simulink model "ButtonLogic"  (R2023b)
settings: Solver=FixedStepDiscrete  StartTime=0.0  StopTime=inf  FixedStep=0.005  RelTol=1e-3  EnableMultiTasking=on
model workspace (MAT data in the model file):
  inSetButton = 0
undefined symbols (not defined in the file or in its folder): eStateName
libraries: simulink x5
(part 2 of 3)

== stateflow chart ButtonLogic/ButtonStates/buttonFlowChart ==
  state Flow [parallel]
    settings: executionOrder=3
    state ButtonTriggeredMenu
      state Menu
        state MainSubMenu
          (history)
          state LapTimer
            en:
            currentState = eStateName.LAP_TIMER;
            state LapTimerEntry
            state GreyedOut
            (default) -> (junction 222)
            LapTimerEntry -> 3149 : SET
            (junction 222) -> LapTimerEntry [order 1] : [rideMode == eRideMode.track]
            (junction 222) -> (junction 225) [order 2]
            (junction 225) -> GreyedOut
          state Motorcycle
            en:
            currentState = eStateName.MOTORCYCLE;
          state BikeInfo
            en:
            currentState = eStateName.BIKE_INFO;
          state TripInfo
            en:
            currentState = eStateName.TRIP_INFO;
          state CruiseControlMain
            en:
            currentState = eStateName.CRUISE_CONTROL;
          state NavigationMain
            en:
            currentState = eStateName.MAIN_NAVIGATION;
            state NavigationGreyedOut
            state NavigationVisible
            (default) -> (junction 1075)
            (junction 1075) -> NavigationGreyedOut [order 1] : [CCU_BT_Status == 0 || rideMode == eRideMode.track]
            (junction 1075) -> (junction 1080) [order 2]
            NavigationVisible -> 3067 : SET
            (junction 1080) -> NavigationVisible
          state HeatedGripsMain
            en:
            currentState = eStateName.HEATED_GRIPS;
          state AudioMain
            en:
            currentState = eStateName.AUDIO;
            state AudioVisible
            state AudioGreyedOut
            (default) -> (junction 1063)
            (junction 1063) -> AudioVisible [order 1] : [CCU_BT_Status == 1]
            AudioVisible -> 3021 : SET
            (junction 1063) -> (junction 1069) [order 2]
            (junction 1069) -> AudioGreyedOut
          state SettingsMain
            en:
            currentState = eStateName.SETTINGS;
            state SettingsGreyedOut
            state SettingsMenu
            (default) -> (junction 1245)
            (junction 1245) -> SettingsGreyedOut [order 1] : [vehSpeed>2.5]
            (junction 1245) -> (junction 1249) [order 2]
            (junction 1249) -> SettingsMenu
            SettingsMenu -> 3009 [order 2] : SET
            SettingsMenu -> 3011 [order 1] : [duration(up && down,msec)>=3000]
          (default) -> (junction 3141)
          (junction 3141) -> LapTimer [order 1] : [rideMode == eRideMode.track]
          (junction 3141) -> Motorcycle [order 2]
          (junction 3145) -> (junction 3141)
          LapTimer -> (junction 3151) [order 2] : UP
          (junction 4100) -> (junction 3151) [order 2]
          (junction 3151) -> (junction 3153)
          (junction 4100) -> LapTimer [order 1] : [rideMode == eRideMode.track]
          LapTimer -> Motorcycle [order 1] : DOWN
          Motorcycle -> (junction 4100) [order 1] : UP
          Motorcycle -> BikeInfo [order 2] : DOWN
          BikeInfo -> Motorcycle [order 1] : UP
          BikeInfo -> TripInfo [order 2] : DOWN
          TripInfo -> BikeInfo [order 1] : UP
          (junction 839) -> TripInfo
          CruiseControlMain -> (junction 839) [order 1] : UP
          (junction 194) -> (junction 839) [order 2]
          TripInfo -> (junction 154) [order 2] : DOWN
          (junction 154) -> CruiseControlMain [order 1] : [ECU_SL_Feature == 1 || ...
              | rideMode != eRideMode.track]
          (junction 194) -> CruiseControlMain [order 1] : [ECU_SL_Feature == 1]
          NavigationMain -> (junction 194) [order 2] : UP
          (junction 154) -> (junction 157) [order 2]
          (junction 189) -> (junction 194) [order 2]
          CruiseControlMain -> (junction 157) [order 2] : DOWN
          (junction 157) -> NavigationMain [order 1] : [CCU_Status == eCCUStatus.installed && CCU_TbT_Navigation_Feature == 1]
          (junction 189) -> NavigationMain [order 1] : [CCU_Status == eCCUStatus.installed && CCU_TbT_Navigation_Feature == 1]
          (junction 157) -> (junction 163) [order 2]
          HeatedGripsMain -> (junction 189) [order 2] : UP
          (junction 186) -> (junction 189) [order 2]
          NavigationMain -> (junction 163) [order 1] : DOWN
          (junction 163) -> HeatedGripsMain [order 1] : [Heated_Grips == 1 ]
              |  //Menu Settings/Heating/Heating Grip == Not available]
          (junction 163) -> (junction 171) [order 2]
          (junction 186) -> HeatedGripsMain [order 1] : [Heated_Grips == 1 ]
          Flow.ButtonTriggeredMenu.Menu.MainSubMenu.AudioMain -> (junction 186) [order 2] : UP
          (junction 183) -> (junction 186) [order 2] : [CCU_Status == eCCUStatus.notInstalled || CCU_Music_Feature == 0]
          HeatedGripsMain -> (junction 171) [order 1] : DOWN
          (junction 171) -> Flow.ButtonTriggeredMenu.Menu.MainSubMenu.AudioMain [order 1] : [CCU_Status == eCCUStatus.installed && CCU_Music_Feature == 1]
          (junction 171) -> (junction 177) [order 2]
          (junction 183) -> Flow.ButtonTriggeredMenu.Menu.MainSubMenu.AudioMain [order 1] : [CCU_Status == eCCUStatus.installed && CCU_Music_Feature == 1]
          (junction 4104) -> (junction 183) [order 2]
          (junction 181) -> (junction 183)
          Flow.ButtonTriggeredMenu.Menu.MainSubMenu.AudioMain -> (junction 177) [order 1] : DOWN
          (junction 3153) -> (junction 4104)
          (junction 4104) -> SettingsMain [order 1] : [vehSpeed<2.5]
          (junction 177) -> SettingsMain [order 1] : [vehSpeed<=2.5]
          SettingsMain -> (junction 181) [order 1] : UP
          (junction 177) -> (junction 3145) [order 2]
          SettingsMain -> (junction 3145) [order 2] : DOWN
        state Lap_TimerV1 [commented out]
          state LapTimerLoop [commented out]
            en:
            currentState = eStateName.RESET_LAPS;
            roundTimer = roundTimerData_arr[roundTimeCounter];
          state ResetLaps [commented out]
            state Keep [commented out]
              en:
              currentState = eStateName.KEEP;
            state Reset [commented out]
              en:
              currentState = eStateName.RESET;
              roundTimerData_arr[roundTimeCounter] =0;
              //updateRoundTimeData();
            (default) -> Flow.ButtonTriggeredMenu.Menu.Lap_TimerV1.ResetLaps.Keep [commented out]
            Flow.ButtonTriggeredMenu.Menu.Lap_TimerV1.ResetLaps.Keep -> Flow.ButtonTriggeredMenu.Menu.Lap_TimerV1.ResetLaps.Reset [commented out] : DOWN
            Flow.ButtonTriggeredMenu.Menu.Lap_TimerV1.ResetLaps.Reset -> Flow.ButtonTriggeredMenu.Menu.Lap_TimerV1.ResetLaps.Keep [commented out] : UP
          (default) -> Flow.ButtonTriggeredMenu.Menu.Lap_TimerV1.LapTimerLoop [commented out] : {roundTimeCounter = 0;
              | copyRoundTimeData();
              | updateRoundTimeData();}
          Flow.ButtonTriggeredMenu.Menu.Lap_TimerV1.LapTimerLoop -> (junction 237) [commented out] : DOWN
          (junction 237) -> (junction 240) [commented out] : [roundTimeCounter < BLU_MaxRndTimeLoopLim]
          (junction 240) -> (junction 239) [commented out] : {roundTimeCounter++;}
          (junction 237) -> (junction 239) [commented out]
          (junction 239) -> Flow.ButtonTriggeredMenu.Menu.Lap_TimerV1.LapTimerLoop [commented out]
          Flow.ButtonTriggeredMenu.Menu.Lap_TimerV1.LapTimerLoop -> (junction 245) [commented out] : UP
          (junction 245) -> (junction 247) [commented out] : [roundTimeCounter>0]
          (junction 247) -> (junction 249) [commented out] : {roundTimeCounter--;}
          (junction 245) -> (junction 249) [commented out]
          (junction 249) -> Flow.ButtonTriggeredMenu.Menu.Lap_TimerV1.LapTimerLoop [commented out]
          Flow.ButtonTriggeredMenu.Menu.Lap_TimerV1.LapTimerLoop -> Flow.ButtonTriggeredMenu.Menu.Lap_TimerV1.ResetLaps [commented out] : SET
          Flow.ButtonTriggeredMenu.Menu.Lap_TimerV1.ResetLaps -> Flow.ButtonTriggeredMenu.Menu.Lap_TimerV1.LapTimerLoop [commented out] : EXIT
        state NoQS
          en:
          QuickSelectorDbg = 1;
        state Lap_TimerV2
          state LapTimerLoop
            en:
            currentState = eStateName.RESET_LAPS;
          state RoundTimerMenu
            en:
            currentState = eStateName.RESET_LAPS_RND_TMR;
          state ResetLaps
            state ResetLapsMenu
              state Keep
                en:
                currentState = eStateName.RESETLAPS_KEEP;
              state Reset
                en:
                currentState = eStateName.RESETLAPS_RESET;
                //updateRoundTimeData();
              (default) -> Flow.ButtonTriggeredMenu.Menu.Lap_TimerV2.ResetLaps.ResetLapsMenu.Keep
              Flow.ButtonTriggeredMenu.Menu.Lap_TimerV2.ResetLaps.ResetLapsMenu.Keep -> Flow.ButtonTriggeredMenu.Menu.Lap_TimerV2.ResetLaps.ResetLapsMenu.Reset [order 1] : DOWN || UP
              Flow.ButtonTriggeredMenu.Menu.Lap_TimerV2.ResetLaps.ResetLapsMenu.Reset -> Flow.ButtonTriggeredMenu.Menu.Lap_TimerV2.ResetLaps.ResetLapsMenu.Keep [order 1] : DOWN || UP
            Flow.ButtonTriggeredMenu.Menu.Lap_TimerV2.ResetLaps.ResetLapsMenu.Keep -> (junction 3560) [order 2] : SET
            (junction 3560) -> 3554
            ResetLapsMenu -> 3554 : EXIT
            (junction 3565) -> 3554
            Flow.ButtonTriggeredMenu.Menu.Lap_TimerV2.ResetLaps.ResetLapsMenu.Reset -> (junction 3565) [order 2] : SET
                | {BLU_FnRLResetRndTmr();}
          (junction 4160) -> 3133
          RoundTimerMenu -> (junction 4160) [order 3] : EXIT
          Flow.ButtonTriggeredMenu.Menu.Lap_TimerV2.LapTimerLoop -> 3133 [order 2] : EXIT
          (default) -> (junction 3138)
          (junction 3138) -> Flow.ButtonTriggeredMenu.Menu.Lap_TimerV2.LapTimerLoop : {roundTimeCounter = 0;
              | copyRoundTimeData();
              | updateRoundTimeData();}
          3135 -> (junction 3138)
          (junction 4150) -> Flow.ButtonTriggeredMenu.Menu.Lap_TimerV2.LapTimerLoop
          (junction 4058) -> (junction 4150) [order 2]
          RoundTimerMenu -> (junction 4058) [order 1] : UP
          (junction 4058) -> (junction 4060) [order 1] : [BLU_RND_TMR_LOOP ==1]
          Flow.ButtonTriggeredMenu.Menu.Lap_TimerV2.LapTimerLoop -> (junction 4257) [order 4] : UP
          (junction 4257) -> RoundTimerMenu : [BLU_RND_TMR_LOOP ==1]
              | {BLU_FnLapTmrScrllUP();}
          (junction 4065) -> (junction 4058) [order 2]
          (junction 4060) -> (junction 4062) : {BLU_FnRLRndTmrUp();}
          (junction 4062) -> RoundTimerMenu
          Flow.ButtonTriggeredMenu.Menu.Lap_TimerV2.LapTimerLoop -> Flow.ButtonTriggeredMenu.Menu.Lap_TimerV2.ResetLaps [order 1] : SET
          3555 -> Flow.ButtonTriggeredMenu.Menu.Lap_TimerV2.LapTimerLoop
          Flow.ButtonTriggeredMenu.Menu.Lap_TimerV2.LapTimerLoop -> (junction 4052) [order 3] : DOWN
          (junction 4063) -> (junction 4062) : {BLU_FnRLRndTmrDwn();}
          (junction 4065) -> (junction 4063) [order 1] : [BLU_RND_TMR_LOOP ==1]
          RoundTimerMenu -> (junction 4065) [order 2] : DOWN
          (junction 4052) -> RoundTimerMenu : [BLU_RND_TMR_LOOP ==1]
              | {BLU_FnLapTmrScrllDOWN();}
        state MotorCycleSubMenu
          state MotorCycleSubMenu1
            (history)
            state RideMode
              en:
              currentState = eStateName.MOTORCYCLE_RIDEMODE;
            state ABS
              en:
              currentState = eStateName.MOTORCYCLE_ABS;
            state MTC
              en:
              currentState = eStateName.MOTORCYCLE_MTC;
            state LaunchControl
              en:
              currentState = eStateName.MOTORCYCLE_LAUNCHCONTROL;
            (junction 3116) -> RideMode
            (junction 3124) -> (junction 3116)
            RideMode -> (junction 3119) [order 3] : UP
            (junction 3119) -> (junction 3121)
            RideMode -> ABS [order 1] : DOWN
            ABS -> RideMode [order 1] : UP
            (junction 4113) -> ABS
            (junction 4111) -> (junction 4113) [order 2]
            MTC -> (junction 4113) [order 1] : UP
            ABS -> (junction 4107) [order 3] : DOWN
            (junction 4107) -> MTC [order 1] : [ABS_TC_MTC_Mode_Feature !=eTCMode.TCMode_OFF]
            (junction 3121) -> (junction 4246)
            (junction 4107) -> (junction 1612) [order 2]
            MTC -> (junction 1612) [order 2] : DOWN
            (junction 4111) -> MTC [order 1] : [ABS_TC_MTC_Mode_Feature !=eTCMode.TCMode_OFF]
            (junction 4246) -> (junction 4111) [order 2]
            (junction 4246) -> (junction 4248) [order 1] : [rideMode == eRideMode.rain && ...
                | ABS_Launch_Control_Feature == 1]
            LaunchControl -> (junction 4111) [order 1] : UP
            (junction 1612) -> LaunchControl [order 1] : [rideMode == eRideMode.rain && ...
                | ABS_Launch_Control_Feature == 1]
            (junction 1612) -> (junction 3551) [order 2]
            (junction 4248) -> LaunchControl
            (junction 3551) -> (junction 3124)
            LaunchControl -> (junction 3551) [order 3] : DOWN
          state RideModeSubMenu
            state RideModeSubMenu1
              (history)
              state Track
                en:
                currentState = eStateName.MC_RIDEMODE_TRACK;
              state Street
                en:
                currentState = eStateName.MC_RIDEMODE_STREET;
              state Rain
                en:
                currentState = eStateName.MC_RIDEMODE_RAIN;
              Track -> (junction 3105) [order 1]
              (junction 3112) -> Track
              (junction 3105) -> (junction 3107) [order 2] : DOWN
              (junction 3110) -> (junction 3112)
              Track -> Street [order 2] : UP
              Street -> Track [order 3] : DOWN
              Rain -> Street [order 1] : DOWN
              Street -> Rain [order 2] : UP
              (junction 3107) -> Rain
              Rain -> (junction 3110) [order 3] : UP
            state TrackCloseThrottle
              en:
              currentState = eStateName.MC_CLOSETHROTTLE;
            state KillSwitch
              en:
              currentState = eStateName.MC_DEACTIVATE_KILLSWITCH;
            state StreetCloseThrottle
              en:
              currentState = eStateName.MC_CLOSETHROTTLE;
            state RainCloseThrottle
              en:
              currentState = eStateName.MC_CLOSETHROTTLE;
            (junction 3105) -> (junction 1639) [order 1] : SET
            (junction 1639) -> (junction 2456) [order 1] : [killSwitch == eSwitch.closed]
            (junction 2456) -> TrackCloseThrottle : {DASH_TC_Mode_Request = 0;
                | DASH_Drive_Mode_Request = 0;}
            (junction 1639) -> KillSwitch [order 2]
            TrackCloseThrottle -> (junction 1665) [order 2] : after(5,sec)
            TrackCloseThrottle -> (junction 1664) [order 1] : after(500,msec)
            KillSwitch -> (junction 1659) : [after(1,sec)]
            (junction 1665) -> (junction 1659)
            (junction 1664) -> (junction 1665) : [ABS_TC_Mode_Response == 0 && ...
                | ECU_Drive_Mode_Response == 0]
                | {rideMode = eRideMode.track;}
            (junction 1659) -> (junction 1680)
            (junction 1651) -> KillSwitch [order 2]
            2646 -> (junction 2143)
            (junction 2143) -> Street
            2655 -> (junction 2143)
            Street -> (junction 1651) [order 1] : SET
            (junction 1651) -> (junction 2458) [order 1] : [killSwitch == eSwitch.closed]
            (junction 2458) -> StreetCloseThrottle : {DASH_TC_Mode_Request = 0;
                | DASH_Drive_Mode_Request = 0;}
            StreetCloseThrottle -> (junction 2611) [order 1] : after(500,msec)
            (junction 1654) -> (junction 1651) [order 2]
            (junction 2611) -> (junction 2615) : [ABS_TC_Mode_Response == 0 && ...
                | ECU_Drive_Mode_Response == 0]
                | {rideMode = eRideMode.street;}
            StreetCloseThrottle -> (junction 1677) [order 2] : after(5,sec)
            (junction 1677) -> (junction 1680)
            (junction 2615) -> (junction 1677)
            (junction 1680) -> 2653
            RainCloseThrottle -> (junction 1677) [order 2] : after(5,sec)
            (junction 2613) -> (junction 2615) : [ABS_TC_Mode_Response == 2 && ...
                | ECU_Drive_Mode_Response == 2]
                | {rideMode = eRideMode.rain;}
            RainCloseThrottle -> (junction 2613) [order 1] : after(500,msec)
            Rain -> (junction 1654) [order 2] : SET
            (junction 1654) -> (junction 2459) [order 1] : [killSwitch == eSwitch.closed]
            (junction 2459) -> RainCloseThrottle : {DASH_TC_Mode_Request = 2;
                | DASH_Drive_Mode_Request = 2;}
            RideModeSubMenu1 -> 2653 : EXIT
          state ABSSubMenu
            state ABSMenu1
              (history)
              state ABSRoad
                en:
                currentState = eStateName.ABS_ROAD;
              state ABSSuperMoto
                en:
                currentState = eStateName.ABS_SUPERMOTO;
              ABSRoad -> (junction 1706) [order 1] : DOWN || UP
              ABSSuperMoto -> ABSRoad [order 1] : DOWN || UP
              (junction 1706) -> ABSSuperMoto : [ABS_Mode_Feature == 1]
            state SetABStoRoad
              en:
              DASH_ABS_Mode_Request = eABSMode.road;
            state SetABStoSupermoto
              en:
              DASH_ABS_Mode_Request = eABSMode.supermoto;
            2154 -> (junction 2156)
            SetABStoRoad -> (junction 2669) [order 1] : after(500,msec)
            ABSRoad -> SetABStoRoad [order 2] : SET
            (junction 2156) -> ABSRoad
            (junction 2669) -> (junction 2550) : [ABS_ABS_Mode_Response == eABSMode.road]
            2642 -> (junction 2156)
            SetABStoRoad -> (junction 2553) [order 2] : after(5,sec)
            (junction 2550) -> (junction 2553)
            ABSMenu1 -> 2636 : EXIT
            (junction 2553) -> 2636
            SetABStoSupermoto -> (junction 2553) [order 2] : after(5,sec)
            (junction 2671) -> (junction 2550) : [ABS_ABS_Mode_Response == eABSMode.supermoto]
            SetABStoSupermoto -> (junction 2671) [order 1] : after(500,msec)
            ABSSuperMoto -> SetABStoSupermoto [order 2] : SET
          state MTCSubMenu
            state MTCMenuOptions
              (history)
              state MTC_Off
                en:
                currentState = eStateName.MTCMODE_OFF;
              state MTC_On
                en:
                currentState = eStateName.MTCMODE_ON;
              (default) -> MTC_Off
              MTC_Off -> MTC_On [order 1] : DOWN || UP
              MTC_On -> MTC_Off [order 1] : DOWN || UP
            state MTC_Message
              en:
              currentState = eStateName.MTC_KEEP_OFF_PRESS;
            state MTC_Release
              en:
              currentState = eStateName.MTC_OFF_RELEASE;
            state MTC_Message1
              en:
              currentState = eStateName.MTC_KEEP_ON_PRESS;
            state MTC_Release1
              en:
              currentState = eStateName.MTC_ON_RELEASE;
            2163 -> (junction 2165)
            (junction 2165) -> (junction 1732)
            (junction 1732) -> (junction 1734) [order 1] : [ABS_TC_MTC_Mode_Feature == eTCMode.TCMode_TC || ...
                | ABS_TC_MTC_Mode_Feature == eTCMode.TCMode_TC_Demo ]
            (junction 1732) -> (junction 1739) [order 2]
            2630 -> (junction 2165)
            (junction 1734) -> (junction 1741) : {currentState = eStateName.MTCMODE_TC;}
            (junction 1739) -> (junction 1741) : {currentState = eStateName.MTCMODE_MTC;}
            (junction 1741) -> MTCMenuOptions
            MTC_Off -> MTC_Message [order 2] : [set]
            MTC_Message -> MTC_Release [order 2] : after(3,sec)
            MTC_Message -> (junction 2545) [order 1] : [!set]
            MTC_Release -> (junction 1761) : [!set]
                | {DASH_MTC_Off_Switch = eButton.pressed;}
            MTCMenuOptions -> 2623 : EXIT
            (junction 2545) -> 2623
            (junction 1761) -> (junction 2545)
            MTC_Message1 -> (junction 2545) [order 1] : [!set]
            MTC_Release1 -> (junction 1761) : [!set]
                | {DASH_MTC_Off_Switch = eButton.released;}
            MTC_On -> MTC_Message1 [order 2] : [set]
            MTC_Message1 -> MTC_Release1 [order 2] : after(3,sec)
          state LaunchControlSubMenu
            state LaunchControlSubMenu1
              (history)
              state LaunchControlON
                en:
                currentState = eStateName.MC_LAUNCHCONTROL_ON;
              state LaunchControlOFF
                en:
                currentState = eStateName.MC_LAUNCHCONTROL_OFF;
              LaunchControlON -> LaunchControlOFF [order 2] : DOWN || UP
              LaunchControlOFF -> LaunchControlON [order 1] : DOWN || UP
            2616 -> LaunchControlON
            LaunchControlON -> (junction 1785) [order 1] : SET
            (junction 1785) -> (junction 1789) : {BLU_FnLaunchControlON();}
            (junction 1787) -> (junction 1789) : {BLU_FnLaunchControlOFF();}
            (junction 1789) -> 2618
            LaunchControlOFF -> (junction 1787) [order 2] : SET
            LaunchControlSubMenu1 -> 2618 : EXIT
          3127 -> (junction 3116)
          RideMode -> 2656 [order 2] : SET
          2649 -> 2647
          2654 -> (junction 2659)
          (junction 2659) -> (junction 2639)
          ABS -> 2643 [order 2] : SET
          2287 -> 2155
          2637 -> (junction 2639)
          (junction 2639) -> (junction 2633)
          MotorCycleSubMenu1 -> 3130 : EXIT
          (junction 1728) -> 2631 : [ABS_TC_MTC_Mode_Feature == eTCMode.TCMode_TC || ...
              | ABS_TC_MTC_Mode_Feature == eTCMode.TCMode_MTC || ...
              | ABS_TC_MTC_Mode_Feature == eTCMode.TCMode_TC_Demo || ...
              | ABS_TC_MTC_Mode_Feature == eTCMode.TCMode_MTC_Demo ]
          MTC -> (junction 1728) [order 3] : SET
          2290 -> 2164
          2624 -> (junction 2633)
          (junction 2633) -> (junction 2662)
          (junction 2662) -> MotorCycleSubMenu1
          2619 -> (junction 2662)
          LaunchControl -> 2617 [order 2] : SET
        state BikeInfoSubMenu
          state BikeInfoSubMenuMain
            state WaterTemp
              en:
              currentState = eStateName.WATER_TEMPERATURE;
            state FuelRange
              en:
              currentState = eStateName.FUEL_RANGE;
            state Battery
              en:
              currentState = eStateName.BATTERY;
            state Odometer
              en:
              currentState = eStateName.ODOMETER;
            state Service
              en:
              currentState = eStateName.SERVICE;
            state Warnings
              en:
              currentState = eStateName.WARNINGS;
            (default) -> (junction 3096)
            WaterTemp -> (junction 3088) [order 2] : UP
            (junction 3096) -> WaterTemp
            (junction 3094) -> (junction 3096)
            (junction 3088) -> (junction 3090)
            WaterTemp -> FuelRange [order 1] : DOWN
            FuelRange -> WaterTemp [order 2] : UP
            FuelRange -> Battery [order 1] : DOWN
            Battery -> FuelRange [order 2] : UP
            Battery -> Odometer [order 1] : DOWN
            Odometer -> Battery [order 2] : UP
            Odometer -> Service [order 1] : DOWN
            Service -> Odometer [order 2] : UP
            Service -> Warnings [order 1] : DOWN
            Warnings -> Service [order 1] : UP
            (junction 3090) -> Warnings
            Warnings -> (junction 3094) [order 3] : DOWN
          state WarningsSubMenu
            en:
            currentState = eStateName.WARNINGS_MENU;
          3099 -> BikeInfoSubMenuMain
          4047 -> BikeInfoSubMenuMain
          BikeInfoSubMenuMain -> 3102 : EXIT
          WarningsSubMenu -> (junction 454) [order 2] : UP
          (junction 454) -> (junction 456) : {BLU_FnBIWarningsUp();}
          WarningsSubMenu -> (junction 3090) [order 1] : EXIT
          (junction 456) -> WarningsSubMenu
          (junction 460) -> (junction 456) : {BLU_FnBIWarningsDwn();}
          Warnings -> WarningsSubMenu [order 2] : SET
          WarningsSubMenu -> (junction 460) [order 3] : DOWN
        state TripInfoSubMenu
          state TripInfoSubMenuMain
            (history)
            state TRIP1
              en:
              currentState = eStateName.TRIP_INFO_TRIP_1;
            state TRIP2
              en:
              currentState = eStateName.TRIP_INFO_TRIP_2;
            TRIP1 -> TRIP2 [order 1] : DOWN || UP
            TRIP2 -> TRIP1 [order 1] : DOWN || UP
          state Trip1
            state Trip1SubMenu
              state SetAsOverview
                en:
                currentState = eStateName.TRIP_1_SET_AS_OVERVIEW;
              state ResetTrip
                en:
                currentState = eStateName.TRIP_1_RESET_TRIP;
              Flow.ButtonTriggeredMenu.Menu.TripInfoSubMenu.Trip1.Trip1SubMenu.SetAsOverview -> (junction 2202) [order 2] : SET
                  | {BLU_FnTISetAsOvwTrip1();}
              (junction 2202) -> (junction 398)
              Flow.ButtonTriggeredMenu.Menu.TripInfoSubMenu.Trip1.Trip1SubMenu.SetAsOverview -> Flow.ButtonTriggeredMenu.Menu.TripInfoSubMenu.Trip1.Trip1SubMenu.ResetTrip [order 1] : DOWN || UP
              Flow.ButtonTriggeredMenu.Menu.TripInfoSubMenu.Trip1.Trip1SubMenu.ResetTrip -> Flow.ButtonTriggeredMenu.Menu.TripInfoSubMenu.Trip1.Trip1SubMenu.SetAsOverview [order 1] : DOWN || UP
              Flow.ButtonTriggeredMenu.Menu.TripInfoSubMenu.Trip1.Trip1SubMenu.ResetTrip -> (junction 398) [order 2] : SET
                  | {BLU_FnTIResetTrip1();}
            2176 -> (junction 2175)
            (junction 2175) -> Flow.ButtonTriggeredMenu.Menu.TripInfoSubMenu.Trip1.Trip1SubMenu.SetAsOverview
            (default) -> (junction 2175)
            (junction 398) -> 3935
            Trip1SubMenu -> 3935 : EXIT
          state Trip2
            state Trip2SubMenu
              state SetAsOverview
                en:
                currentState = eStateName.TRIP_2_SET_AS_OVERVIEW;
              state ResetTrip
                en:
                currentState = eStateName.TRIP_2_RESET_TRIP;
              Flow.ButtonTriggeredMenu.Menu.TripInfoSubMenu.Trip2.Trip2SubMenu.SetAsOverview -> (junction 410) [order 2] : SET
                  | {BLU_FnTISetAsOvwTrip2();}
              (junction 2205) -> (junction 410)
              Flow.ButtonTriggeredMenu.Menu.TripInfoSubMenu.Trip2.Trip2SubMenu.SetAsOverview -> Flow.ButtonTriggeredMenu.Menu.TripInfoSubMenu.Trip2.Trip2SubMenu.ResetTrip [order 1] : DOWN || UP
              Flow.ButtonTriggeredMenu.Menu.TripInfoSubMenu.Trip2.Trip2SubMenu.ResetTrip -> Flow.ButtonTriggeredMenu.Menu.TripInfoSubMenu.Trip2.Trip2SubMenu.SetAsOverview [order 1] : DOWN || UP
              Flow.ButtonTriggeredMenu.Menu.TripInfoSubMenu.Trip2.Trip2SubMenu.ResetTrip -> (junction 2205) [order 2] : SET
                  | {BLU_FnTIResetTrip2();}
            (junction 3943) -> 3940
            Trip2SubMenu -> 3940 : EXIT
            (junction 410) -> (junction 3943)
            2209 -> (junction 2212)
            (default) -> (junction 2212)
            (junction 2212) -> Flow.ButtonTriggeredMenu.Menu.TripInfoSubMenu.Trip2.Trip2SubMenu.SetAsOverview
          TRIP1 -> Trip1 [order 2] : SET
          2269 -> 2177
          3082 -> TRIP1
          3936 -> (junction 3946)
          (junction 3946) -> TripInfoSubMenuMain
          3941 -> (junction 3946)
          TripInfoSubMenuMain -> 3080 : EXIT
          TRIP2 -> Trip2 [order 2] : SET
          2273 -> 2210
        state CruiseCtrlSubMenu
          note: Invisible when ECU_CC_Feature == 0
          note: Invisible when ECU_CC_Feature == 1
          state Mode
            en:
            currentState = eStateName.MODE_CC;
          state SpeedLimiter
            en:
            currentState = eStateName.SPEED_LIMITER;
          state SpeedLimiterSubMenu
            (history)
            state SL_ON
              en:
              currentState = eStateName.SPEED_LIMITER_ON;
            state SL_OFF
              en:
              currentState = eStateName.SPEED_LIMITER_OFF;
            (default) -> SL_ON
            SL_ON -> SL_OFF [order 1] : DOWN || UP
            SL_OFF -> SL_ON [order 1] : DOWN || UP
          state ECU_SL_StatusCheck1
            state DashSLONCheck
              en:
              currentState = eStateName.SPEED_LIMITER_ONCHECK;
            state DashSLOFFCheck
              en:
              currentState = eStateName.SPEED_LIMITER_OFFCHECK;
          state ModeSubMenu
            (history)
            state CruiseControlMode1
              en:
              currentState = eStateName.CRUISE_CONTROL_MODE;
            state SpeedLimiterMode
              en:
              currentState = eStateName.SPEED_LIMITER_MODE;
            (default) -> CruiseControlMode1
            CruiseControlMode1 -> SpeedLimiterMode [order 1] : DOWN || UP
            SpeedLimiterMode -> CruiseControlMode1 [order 1] : DOWN || UP
          state ECU_SL_StatusCheck2
            state DashCruiseCtrlChck
              en:
              currentState = eStateName.CRUISE_CONTROL_CHECK;
            state DashSpeedLmtrChck
              en:
              currentState = eStateName.SPEED_LIMITER_MODE_CHECK;
          3072 -> (junction 481)
          (default) -> (junction 481)
          (junction 481) -> SpeedLimiter [order 2]
          (junction 481) -> Mode [order 1] : [ECU_CC_Feature == 1]
          2266 -> (junction 481)
          SpeedLimiter -> SpeedLimiterSubMenu [order 1] : SET
          (junction 4251) -> SpeedLimiter
          SpeedLimiter -> 3070 [order 2] : EXIT
          Mode -> (junction 490) [order 1] : EXIT
          (junction 4253) -> Mode
          Mode -> ModeSubMenu [order 2] : SET
          (junction 4189) -> (junction 4185)
          (junction 4185) -> (junction 4169)
          (junction 4169) -> (junction 4253)
          (junction 490) -> 3070
          ECU_SL_StatusCheck2 -> (junction 4185) [order 2] : [after(5,sec)]
          ECU_SL_StatusCheck2 -> (junction 4189) [order 1] : EXIT
          ModeSubMenu -> (junction 4253) : EXIT
          (junction 550) -> (junction 4169)
          SpeedLimiterSubMenu -> (junction 4251) : EXIT
          (junction 4192) -> (junction 4251)
          (junction 4194) -> (junction 4192)
          (junction 512) -> (junction 4251)
          ECU_SL_StatusCheck1 -> (junction 4192) [order 2] : [after(5,sec)]
          ECU_SL_StatusCheck1 -> (junction 4194) [order 1] : EXIT
          CruiseControlMode1 -> DashCruiseCtrlChck [order 2] : SET
              | {DASH_SL_Switch =1;}
          SL_ON -> DashSLONCheck [order 2] : SET
              | {DASH_SL_Switch =1;}
          DashCruiseCtrlChck -> (junction 550) : [ ECU_SL_Status == 0]
              | {BLU_FnCCSwtONCrsCtrl();}
          DashSLONCheck -> (junction 512) : [ ECU_SL_Status == 1]
              | {BLU_FnCCSwtONSpdLmtr();}
          (junction 540) -> (junction 550)
          (junction 523) -> (junction 512)
          SL_OFF -> DashSLOFFCheck [order 2] : SET
              | {DASH_SL_Switch =1;}
          SpeedLimiterMode -> DashSpeedLmtrChck [order 2] : SET
              | {DASH_SL_Switch =1;}
          DashSLOFFCheck -> (junction 523) : [ ECU_SL_Status == 0]
              | {BLU_FnCCSwtOFFSpdLmtr();}
          DashSpeedLmtrChck -> (junction 540) : [ ECU_SL_Status == 1]
              | {BLU_FnCCSwtONSpdLmtr();}
        state NavigationVolSubMenu
          state NavGroup
            (history)
            state Volume
              en:
              currentState = eStateName.NAVIGATION_VOLUME;
            state Navigation
              en:
              currentState = eStateName.NAVIGATION;
            (default) -> Volume
            Volume -> Navigation [order 1] : DOWN || UP
            Navigation -> Volume [order 1] : DOWN || UP
          state VolumeSubMenu
            en:
            currentState = eStateName.NAVIGATION_VOL_SUB_MN;
          state NavigationSubMenu
            (history)
            state Nav_ON
              en:
              currentState = eStateName.NAVIGATION_ON;
            state Nav_OFF
              en:
              currentState = eStateName.NAVIGATION_OFF;
            (default) -> Nav_ON
            Nav_ON -> Nav_OFF [order 1] : DOWN || UP
            Nav_OFF -> Nav_ON [order 1] : DOWN || UP
          2665 -> (junction 2301)
          VolumeSubMenu -> (junction 566) [order 2] : UP
          (junction 566) -> (junction 568) : {BLU_FnNavVolUp();}
          (junction 568) -> VolumeSubMenu
          (junction 2301) -> NavGroup
          (junction 569) -> (junction 568) : {BLU_FnNavVolDwn();}
          Volume -> VolumeSubMenu [order 2] : SET
          3064 -> (junction 2301)
          VolumeSubMenu -> (junction 569) [order 3] : DOWN
          VolumeSubMenu -> (junction 3057) [order 1] : EXIT
          (junction 3950) -> (junction 3057)
          (junction 3057) -> NavGroup
          (junction 2393) -> (junction 3950)
          NavigationSubMenu -> (junction 3057) : EXIT
          NavGroup -> 3062 : EXIT
          Navigation -> NavigationSubMenu [order 2] : SET
          Nav_ON -> (junction 2389) [order 2] : SET
          (junction 2389) -> (junction 2393) : {navigationStatus = eFeatureStatus.enabled;
              | BLU_FnNavigationStatus(navigationStatus);}
          (junction 2391) -> (junction 2393) : {navigationStatus = eFeatureStatus.disabled;
              | BLU_FnNavigationStatus(navigationStatus);}
          Nav_OFF -> (junction 2391) [order 2] : SET
        state HeatedGripsSubMenu
          state HeatedGripsMenuGrp
            (history)
            state HeatedGripsOFF
              en:
              currentState = eStateName.HEATED_GRIPS_OFF;
              HeatedGripsMode = eHeatedGripsMode.OFF;
            state HeatedGripsMAXIMUM
              en:
              currentState = eStateName.HEATED_GRIPS_MAXIMUM;
              HeatedGripsMode = eHeatedGripsMode.MAXIMUM;
            state HeatedGripsMEDIUM
              en:
              currentState = eStateName.HEATED_GRIPS_MEDIUM;
              HeatedGripsMode = eHeatedGripsMode.MEDIUM;
            state HeatedGripsMINIMUM
              en:
              currentState = eStateName.HEATED_GRIPS_MINIMUM;
              HeatedGripsMode = eHeatedGripsMode.MINIMUM;
            HeatedGripsOFF -> (junction 3042) [order 2] : UP
            (junction 3042) -> (junction 3044)
            (junction 3049) -> HeatedGripsOFF
            (junction 3047) -> (junction 3049)
            HeatedGripsOFF -> HeatedGripsMAXIMUM [order 1] : DOWN
            HeatedGripsMAXIMUM -> HeatedGripsOFF [order 1] : UP
            HeatedGripsMAXIMUM -> HeatedGripsMEDIUM [order 2] : DOWN
            HeatedGripsMEDIUM -> HeatedGripsMAXIMUM [order 1] : UP
            HeatedGripsMEDIUM -> HeatedGripsMINIMUM [order 2] : DOWN
            HeatedGripsMINIMUM -> HeatedGripsMEDIUM [order 1] : UP
            (junction 3044) -> HeatedGripsMINIMUM
            HeatedGripsMINIMUM -> (junction 3047) [order 2] : DOWN
          2319 -> (junction 3049)
          3052 -> (junction 3049)
          HeatedGripsMenuGrp -> 3055 [order 1] : EXIT
          (junction 3813) -> 3055 : {BLU_FnSetHeatedGripsMode(HeatedGripsMode);}
          HeatedGripsMenuGrp -> (junction 3813) [order 2] : SET
        state AudioSubMenu
          state AudioMain
            en:
            currentState = eStateName.AUDIO_SUB_MENU;
          Flow.ButtonTriggeredMenu.Menu.AudioSubMenu.AudioMain -> (junction 622) [order 1] : SET
          (junction 622) -> (junction 624) : {BLU_FnAudioTglPlayPause();}
          (junction 624) -> (junction 634)
          2221 -> (junction 2223)
          Flow.ButtonTriggeredMenu.Menu.AudioSubMenu.AudioMain -> (junction 626) [order 2] : longUP
          (junction 626) -> (junction 634) : {BLU_FnAudioVolUp();}
          (junction 634) -> (junction 636)
          Flow.ButtonTriggeredMenu.Menu.AudioSubMenu.AudioMain -> (junction 628) [order 3] : longDOWN
          (junction 628) -> (junction 636) : {BLU_FnAudioVolDwn();}
          (junction 2223) -> Flow.ButtonTriggeredMenu.Menu.AudioSubMenu.AudioMain
          3017 -> (junction 2223)
          (junction 636) -> (junction 640)
          Flow.ButtonTriggeredMenu.Menu.AudioSubMenu.AudioMain -> (junction 630) [order 4] : UP
          (junction 630) -> (junction 640) : {BLU_FnAudioNextTrack();}
          (junction 640) -> (junction 643)
          Flow.ButtonTriggeredMenu.Menu.AudioSubMenu.AudioMain -> 3014 [order 6] : EXIT
          Flow.ButtonTriggeredMenu.Menu.AudioSubMenu.AudioMain -> (junction 632) [order 5] : DOWN
          (junction 632) -> (junction 643) : {BLU_FnAudioPrevTrack();}
          (junction 643) -> (junction 646)
          (junction 646) -> Flow.ButtonTriggeredMenu.Menu.AudioSubMenu.AudioMain
        state SettingsSubMenu
          state SettingsMenuScreens
            (history)
            state Favourites
              en:
              currentState = eStateName.FAVOURITES;
            state QuickSelector
              en:
              currentState = eStateName.QUICK_SELECTOR;
            state Connectivity
              en:
              currentState = eStateName.CONNECTIVITY;
            state QuickShifter
              en:
              currentState = eStateName.QUICK_SHIFTER;
            state ShiftLight
              en:
              currentState = eStateName.SHIFT_LIGHT;
            state ClockDate
              en:
              currentState = eStateName.CLOCK_DATE_MN;
            state Units
              en:
              currentState = eStateName.UNITS;
            state Language
              en:
              currentState = eStateName.LANGUAGE;
            state HeatedGripsSettingsMenu
              en:
              currentState = eStateName.HEATED_GRIPS_SETTINGS_MN;
            state ExtraFunctions
              en:
              currentState = eStateName.EXTRA_FUNCTIONS;
            (default) -> (junction 2702)
            (junction 2702) -> Favourites
            (junction 2710) -> (junction 2702)
            Favourites -> (junction 2705) [order 3] : UP
            (junction 2705) -> (junction 2707)
            Favourites -> QuickSelector [order 2] : DOWN
            QuickSelector -> Favourites [order 2] : UP
            (junction 722) -> QuickSelector
            (junction 1102) -> (junction 722) [order 2] : UP
            (junction 719) -> (junction 722) [order 2]
            QuickSelector -> (junction 668) [order 3] : DOWN
            Connectivity -> (junction 1102) [order 1]
            (junction 668) -> Connectivity [order 1] : [CCU_Status == eCCUStatus.installed]
            (junction 668) -> (junction 671) [order 2]
            Connectivity -> (junction 671) [order 2] : DOWN
            (junction 719) -> Connectivity [order 1] : [CCU_Status == eCCUStatus.installed]
            (junction 1134) -> (junction 719) [order 1] : UP
            (junction 711) -> (junction 719) [order 2]
            QuickShifter -> (junction 1134) [order 1]
            (junction 711) -> QuickShifter [order 1] : [ECU_Quickshifter_Feature != 0]
            (junction 671) -> QuickShifter [order 1] : [ECU_Quickshifter_Feature != 0]
            (junction 709) -> (junction 711)
            (junction 671) -> (junction 676) [order 2]
            QuickShifter -> (junction 676) [order 2] : DOWN
            Flow.ButtonTriggeredMenu.Menu.SettingsSubMenu.SettingsMenuScreens.ShiftLight -> (junction 709) [order 2] : UP
            (junction 676) -> Flow.ButtonTriggeredMenu.Menu.SettingsSubMenu.SettingsMenuScreens.ShiftLight
            Flow.ButtonTriggeredMenu.Menu.SettingsSubMenu.SettingsMenuScreens.ShiftLight -> (junction 713) [order 1] : DOWN
            (junction 713) -> ClockDate
            (junction 715) -> Flow.ButtonTriggeredMenu.Menu.SettingsSubMenu.SettingsMenuScreens.ShiftLight [order 1] : UP
            ClockDate -> (junction 715) [order 1]
            ClockDate -> Units [order 2] : DOWN
            Units -> ClockDate [order 1] : UP
            Units -> Language [order 2] : DOWN
            Language -> Units [order 1] : UP
            (junction 706) -> Language
            HeatedGripsSettingsMenu -> (junction 706) [order 1] : UP
            (junction 703) -> (junction 706) [order 2]
            Language -> (junction 699) [order 2] : DOWN
            (junction 699) -> HeatedGripsSettingsMenu [order 1] : [Heated_Grips]
            (junction 699) -> ExtraFunctions [order 2]
            (junction 703) -> HeatedGripsSettingsMenu [order 1] : [Heated_Grips]
            (junction 702) -> (junction 703)
            HeatedGripsSettingsMenu -> ExtraFunctions [order 2] : DOWN
            (junction 2707) -> ExtraFunctions
            ExtraFunctions -> (junction 2710) [order 3] : DOWN
            ExtraFunctions -> (junction 702) [order 1] : UP
          state FavoritesSubMenu
            state FavoritesSlotsMenu
              state FavoritesSlot1
                en:
                currentState = eStateName.FAVORITES_SLOT_1;
              state FavoritesSlot2
                en:
                currentState = eStateName.FAVORITES_SLOT_2;
              state FavoritesSlot3
                en:
                currentState = eStateName.FAVORITES_SLOT_3;
              state FavoritesSlot4
                en:
                currentState = eStateName.FAVORITES_SLOT_4;
              (default) -> (junction 2990)
              (junction 2990) -> FavoritesSlot1
              (junction 2988) -> (junction 2990)
              FavoritesSlot1 -> (junction 2995) [order 3] : UP
              (junction 2995) -> (junction 2997)
              FavoritesSlot1 -> FavoritesSlot2 [order 1] : DOWN
              FavoritesSlot2 -> FavoritesSlot1 [order 2] : UP
              FavoritesSlot2 -> FavoritesSlot3 [order 3] : DOWN
              FavoritesSlot3 -> FavoritesSlot2 [order 1] : UP
              FavoritesSlot3 -> FavoritesSlot4 [order 2] : DOWN
              FavoritesSlot4 -> FavoritesSlot3 [order 1] : UP
              (junction 2997) -> FavoritesSlot4
              FavoritesSlot4 -> (junction 2988) [order 3] : DOWN
            state Slot1Menu
              state Slot1FavoritesMenu
                (history)
                state Slot1TripDistance1
                  en:
                  currentState = eStateName.FAVORITES_TRIP_DISTANCE_1;
                state Slot1AverageSpeed1
                  en:
                  currentState = eStateName.FAVORITES_AVERAGE_SPEED_1;
                state Slot1AverageFuelCons1
                  en:
                  currentState = eStateName.FAVORITES_AVERAGE_FUEL_CONS_1;
                state Slot1TripTime1
                  en:
                  currentState = eStateName.FAVORITES_TRIP_TIME_1;
                state Slot1AverageTripDistance2
                  en:
                  currentState = eStateName.FAVORITES_TRIP_DISTANCE_2;
                state Slot1AverageSpeed2
                  en:
                  currentState = eStateName.FAVORITES_AVERAGE_SPEED_2;
                state Slot1AverageFuelCons2
                  en:
                  currentState = eStateName.FAVORITES_AVERAGE_FUEL_CONS_2;
                state Slot1TripTime2
                  en:
                  currentState = eStateName.FAVORITES_TRIP_TIME_2;
                state Slot1FuelRange
                  en:
                  currentState = eStateName.FAVORITES_FUEL_RANGE;
                state Slot1Date
                  en:
                  currentState = eStateName.FAVORITES_DATE;
                state Slot1Battery
                  en:
                  currentState = eStateName.FAVORITES_BATTERY;
                state Slot1WaterTemperature
                  en:
                  currentState = eStateName.FAVORITES_WATER_TEMPERATURE;
                state Slot1Odometer
                  en:
                  currentState = eStateName.FAVORITES_ODOMETER;
                (default) -> (junction 2864)
                (junction 2864) -> Slot1TripDistance1
                Slot1TripDistance1 -> (junction 2872) [order 2] : UP
                (junction 2866) -> (junction 2864)
                (junction 2872) -> (junction 2876)
                Slot1TripDistance1 -> Slot1AverageSpeed1 [order 1] : DOWN
                Slot1AverageSpeed1 -> Slot1TripDistance1 [order 1] : UP
                Slot1AverageSpeed1 -> Slot1AverageFuelCons1 [order 2] : DOWN
                Slot1AverageFuelCons1 -> Slot1AverageSpeed1 [order 1] : UP
                Slot1AverageFuelCons1 -> Slot1TripTime1 [order 2] : DOWN
                Slot1TripTime1 -> Slot1AverageFuelCons1 [order 1] : UP
                Slot1TripTime1 -> Slot1AverageTripDistance2 [order 2] : DOWN
                Slot1AverageTripDistance2 -> Slot1TripTime1 [order 1] : UP
                Slot1AverageTripDistance2 -> Slot1AverageSpeed2 [order 2] : DOWN
                Slot1AverageSpeed2 -> Slot1AverageTripDistance2 [order 1] : UP
                Slot1AverageSpeed2 -> Slot1AverageFuelCons2 [order 2] : DOWN
                Slot1AverageFuelCons2 -> Slot1AverageSpeed2 [order 1] : UP
                Slot1AverageFuelCons2 -> Slot1TripTime2 [order 2] : DOWN
                Slot1TripTime2 -> Slot1AverageFuelCons2 [order 1] : UP
                Slot1TripTime2 -> Slot1FuelRange [order 2] : DOWN
                Slot1FuelRange -> Slot1TripTime2 [order 1] : UP
                Slot1FuelRange -> Slot1Date [order 2] : DOWN
                Slot1Date -> Slot1FuelRange [order 1] : UP
                Slot1Date -> Slot1Battery [order 2] : DOWN
                Slot1Battery -> Slot1Date [order 1] : UP
                Slot1Battery -> Slot1WaterTemperature [order 2] : DOWN
                Slot1WaterTemperature -> Slot1Battery [order 1] : UP
                Slot1WaterTemperature -> Slot1Odometer [order 2] : DOWN
                Slot1Odometer -> Slot1WaterTemperature [order 1] : UP
                (junction 2876) -> Slot1Odometer
                Slot1Odometer -> (junction 2866) [order 2] : DOWN
              2878 -> Slot1FavoritesMenu
              (junction 4224) -> 2881
              Slot1FavoritesMenu -> (junction 4224) [order 1] : EXIT
              (junction 4222) -> 2881 : {favSlot1Sel = currentState;
                  | BLU_FnSaveSlot1Fav(currentState);}
              (junction 3917) -> (junction 4224) [order 2]
              (junction 3917) -> (junction 4222) [order 1] : [currentState != favSlot2Sel && ...
                  | currentState != favSlot3Sel && ...
                  | currentState != favSlot4Sel ]
              Slot1FavoritesMenu -> (junction 3917) [order 2] : SET
            state Slot2Menu
              state Slot2FavoritesMenu
                (history)
                state Slot2TripDistance1
                  en:
                  currentState = eStateName.FAVORITES_TRIP_DISTANCE_1;
                state Slot2AverageSpeed1
                  en:
                  currentState = eStateName.FAVORITES_AVERAGE_SPEED_1;
                state Slot2AverageFuelCons1
                  en:
                  currentState = eStateName.FAVORITES_AVERAGE_FUEL_CONS_1;
                state Slot2TripTime1
                  en:
                  currentState = eStateName.FAVORITES_TRIP_TIME_1;
                state Slot2AverageTripDistance2
                  en:
                  currentState = eStateName.FAVORITES_TRIP_DISTANCE_2;
                state Slot2AverageSpeed2
                  en:
                  currentState = eStateName.FAVORITES_AVERAGE_SPEED_2;
                state Slot2AverageFuelCons2
                  en:
                  currentState = eStateName.FAVORITES_AVERAGE_FUEL_CONS_2;
                state Slot2TripTime2
                  en:
                  currentState = eStateName.FAVORITES_TRIP_TIME_2;
                state Slot2FuelRange
                  en:
                  currentState = eStateName.FAVORITES_FUEL_RANGE;
                state Slot2Date
                  en:
                  currentState = eStateName.FAVORITES_DATE;
                state Slot2Battery
                  en:
                  currentState = eStateName.FAVORITES_BATTERY;
                state Slot2WaterTemperature
                  en:
                  currentState = eStateName.FAVORITES_WATER_TEMPERATURE;
                state Slot2Odometer
                  en:
                  currentState = eStateName.FAVORITES_ODOMETER;
                (default) -> (junction 2892)
                Slot2TripDistance1 -> (junction 2885) [order 2] : UP
                (junction 2892) -> Slot2TripDistance1
                (junction 2885) -> (junction 2887)
                (junction 2890) -> (junction 2892)
                Slot2TripDistance1 -> Slot2AverageSpeed1 [order 1] : DOWN
                Slot2AverageSpeed1 -> Slot2TripDistance1 [order 1] : UP
                Slot2AverageSpeed1 -> Slot2AverageFuelCons1 [order 2] : DOWN
                Slot2AverageFuelCons1 -> Slot2AverageSpeed1 [order 1] : UP
                Slot2AverageFuelCons1 -> Slot2TripTime1 [order 2] : DOWN
                Slot2TripTime1 -> Slot2AverageFuelCons1 [order 1] : UP
                Slot2TripTime1 -> Slot2AverageTripDistance2 [order 2] : DOWN
                Slot2AverageTripDistance2 -> Slot2TripTime1 [order 1] : UP
                Slot2AverageTripDistance2 -> Slot2AverageSpeed2 [order 2] : DOWN
                Slot2AverageSpeed2 -> Slot2AverageTripDistance2 [order 1] : UP
                Slot2AverageSpeed2 -> Slot2AverageFuelCons2 [order 2] : DOWN
                Slot2AverageFuelCons2 -> Slot2AverageSpeed2 [order 1] : UP
                Slot2AverageFuelCons2 -> Slot2TripTime2 [order 2] : DOWN
                Slot2TripTime2 -> Slot2AverageFuelCons2 [order 1] : UP
                Slot2TripTime2 -> Slot2FuelRange [order 2] : DOWN
                Slot2FuelRange -> Slot2TripTime2 [order 1] : UP
                Slot2FuelRange -> Slot2Date [order 2] : DOWN
                Slot2Date -> Slot2FuelRange [order 1] : UP
                Slot2Date -> Slot2Battery [order 2] : DOWN
                Slot2Battery -> Slot2Date [order 1] : UP
                Slot2Battery -> Slot2WaterTemperature [order 2] : DOWN
                Slot2WaterTemperature -> Slot2Battery [order 1] : UP
                Slot2WaterTemperature -> Slot2Odometer [order 2] : DOWN
                Slot2Odometer -> Slot2WaterTemperature [order 1] : UP
                Slot2Odometer -> (junction 2890) [order 2] : DOWN
                (junction 2887) -> Slot2Odometer
              2896 -> Slot2FavoritesMenu
              (junction 4233) -> 2899
              Slot2FavoritesMenu -> (junction 4233) [order 1] : EXIT
              (junction 4231) -> 2899 : {favSlot1Sel = currentState;
                  | BLU_FnSaveSlot2Fav(currentState);}
              (junction 3922) -> (junction 4233) [order 2]
              (junction 3922) -> (junction 4231) [order 1] : [currentState != favSlot1Sel && ...
                  | currentState != favSlot3Sel && ...
                  | currentState != favSlot4Sel ]
              Slot2FavoritesMenu -> (junction 3922) [order 2] : SET
            state Slot3Menu
              state Slot3FavoritesMenu
                (history)
                state Slot3TripDistance
                  en:
                  currentState = eStateName.FAVORITES_TRIP_DISTANCE_1;
                state Slot3AverageSpeed
                  en:
                  currentState = eStateName.FAVORITES_AVERAGE_SPEED_1;
                state Slot3AverageFuelCons
                  en:
                  currentState = eStateName.FAVORITES_AVERAGE_FUEL_CONS_1;
                state Slot3TripTime
                  en:
                  currentState = eStateName.FAVORITES_TRIP_TIME_1;
                state Slot3AverageTripDistance
                  en:
                  currentState = eStateName.FAVORITES_TRIP_DISTANCE_2;
                state Slot3AverageSpeed1
                  en:
                  currentState = eStateName.FAVORITES_AVERAGE_SPEED_2;
                state Slot3AverageFuelCons1
                  en:
                  currentState = eStateName.FAVORITES_AVERAGE_FUEL_CONS_2;
                state Slot3TripTime2
                  en:
                  currentState = eStateName.FAVORITES_TRIP_TIME_2;
                state Slot3FuelRange
                  en:
                  currentState = eStateName.FAVORITES_FUEL_RANGE;
                state Slot3Date
                  en:
                  currentState = eStateName.FAVORITES_DATE;
                state Slot3Battery
                  en:
                  currentState = eStateName.FAVORITES_BATTERY;
                state Slot3WaterTemperature
                  en:
                  currentState = eStateName.FAVORITES_WATER_TEMPERATURE;
                state Slot3Odometer
                  en:
                  currentState = eStateName.FAVORITES_ODOMETER;
                (default) -> (junction 2914)
                (junction 2914) -> Slot3TripDistance
                Slot3TripDistance -> (junction 2905) [order 2] : UP
                (junction 2912) -> (junction 2914)
                (junction 2905) -> (junction 2907)
                Slot3TripDistance -> Slot3AverageSpeed [order 1] : DOWN
                Slot3AverageSpeed -> Slot3TripDistance [order 1] : UP
                Slot3AverageSpeed -> Slot3AverageFuelCons [order 2] : DOWN
                Slot3AverageFuelCons -> Slot3AverageSpeed [order 1] : UP
                Slot3AverageFuelCons -> Slot3TripTime [order 2] : DOWN
                Slot3TripTime -> Slot3AverageFuelCons [order 1] : UP
                Slot3TripTime -> Slot3AverageTripDistance [order 2] : DOWN
                Slot3AverageTripDistance -> Slot3TripTime [order 1] : UP
                Slot3AverageTripDistance -> Slot3AverageSpeed1 [order 2] : DOWN
                Slot3AverageSpeed1 -> Slot3AverageTripDistance [order 1] : UP
                Slot3AverageSpeed1 -> Slot3AverageFuelCons1 [order 2] : DOWN
                Slot3AverageFuelCons1 -> Slot3AverageSpeed1 [order 1] : UP
                Slot3AverageFuelCons1 -> Slot3TripTime2 [order 2] : DOWN
                Slot3TripTime2 -> Slot3AverageFuelCons1 [order 1] : UP
                Slot3TripTime2 -> Slot3FuelRange [order 2] : DOWN
                Slot3FuelRange -> Slot3TripTime2 [order 1] : UP
                Slot3FuelRange -> Slot3Date [order 2] : DOWN
                Slot3Date -> Slot3FuelRange [order 1] : UP
                Slot3Date -> Slot3Battery [order 2] : DOWN
                Slot3Battery -> Slot3Date [order 1] : UP
                Slot3Battery -> Slot3WaterTemperature [order 2] : DOWN
                Slot3WaterTemperature -> Slot3Battery [order 1] : UP
                Slot3WaterTemperature -> Slot3Odometer [order 2] : DOWN
                Slot3Odometer -> Slot3WaterTemperature [order 1] : UP
                Slot3Odometer -> (junction 2912) [order 2] : DOWN
                (junction 2907) -> Slot3Odometer
              2918 -> Slot3FavoritesMenu
              (junction 4238) -> 2921
              Slot3FavoritesMenu -> (junction 4238) [order 1] : EXIT
              (junction 4236) -> 2921 : {favSlot3Sel = currentState;
                  | BLU_FnSaveSlot3Fav(currentState);}
              (junction 3927) -> (junction 4238) [order 2]
              Slot3FavoritesMenu -> (junction 3927) [order 2] : SET
              (junction 3927) -> (junction 4236) [order 1] : [currentState != favSlot1Sel && ...
                  | currentState != favSlot2Sel && ...
                  | currentState != favSlot4Sel ]
            state Slot4Menu
              state Slot4FavoritesMenu
                (history)
                state Slot4TripDistance
                  en:
                  currentState = eStateName.FAVORITES_TRIP_DISTANCE_1;
                state Slot4AverageSpeed
                  en:
                  currentState = eStateName.FAVORITES_AVERAGE_SPEED_1;
                state Slot4AverageFuelCons
                  en:
                  currentState = eStateName.FAVORITES_AVERAGE_FUEL_CONS_1;
                state Slot4TripTime
                  en:
                  currentState = eStateName.FAVORITES_TRIP_TIME_1;
                state Slot4AverageTripDistance
                  en:
                  currentState = eStateName.FAVORITES_TRIP_DISTANCE_2;
                state Slot4AverageSpeed1
                  en:
                  currentState = eStateName.FAVORITES_AVERAGE_SPEED_2;
                state Slot4AverageFuelCons1
                  en:
                  currentState = eStateName.FAVORITES_AVERAGE_FUEL_CONS_2;
                state Slot4TripTime1
                  en:
                  currentState = eStateName.FAVORITES_TRIP_TIME_2;
                state Slot4FuelRange
                  en:
                  currentState = eStateName.FAVORITES_FUEL_RANGE;
                state Slot4Date
                  en:
                  currentState = eStateName.FAVORITES_DATE;
                state Slot4Battery
                  en:
                  currentState = eStateName.FAVORITES_BATTERY;
                state Slot4WaterTemperature
                  en:
                  currentState = eStateName.FAVORITES_WATER_TEMPERATURE;
                state Slot4Odometer
                  en:
                  currentState = eStateName.FAVORITES_ODOMETER;
                (default) -> (junction 2936)
                (junction 2936) -> Slot4TripDistance
                Slot4TripDistance -> (junction 2937) [order 2] : UP
                (junction 2938) -> (junction 2936)
                (junction 2937) -> (junction 2939)
                Slot4TripDistance -> Slot4AverageSpeed [order 1] : DOWN
                Slot4AverageSpeed -> Slot4TripDistance [order 1] : UP
                Slot4AverageSpeed -> Slot4AverageFuelCons [order 2] : DOWN
                Slot4AverageFuelCons -> Slot4AverageSpeed [order 1] : UP
                Slot4AverageFuelCons -> Slot4TripTime [order 2] : DOWN
                Slot4TripTime -> Slot4AverageFuelCons [order 1] : UP
                Slot4TripTime -> Slot4AverageTripDistance [order 2] : DOWN
                Slot4AverageTripDistance -> Slot4TripTime [order 1] : UP
                Slot4AverageTripDistance -> Slot4AverageSpeed1 [order 2] : DOWN
                Slot4AverageSpeed1 -> Slot4AverageTripDistance [order 1] : UP
                Slot4AverageSpeed1 -> Slot4AverageFuelCons1 [order 2] : DOWN
                Slot4AverageFuelCons1 -> Slot4AverageSpeed1 [order 1] : UP
                Slot4AverageFuelCons1 -> Slot4TripTime1 [order 2] : DOWN
                Slot4TripTime1 -> Slot4AverageFuelCons1 [order 1] : UP
                Slot4TripTime1 -> Slot4FuelRange [order 2] : DOWN
                Slot4FuelRange -> Slot4TripTime1 [order 1] : UP
                Slot4FuelRange -> Slot4Date [order 2] : DOWN
                Slot4Date -> Slot4FuelRange [order 1] : UP
                Slot4Date -> Slot4Battery [order 2] : DOWN
                Slot4Battery -> Slot4Date [order 1] : UP
                Slot4Battery -> Slot4WaterTemperature [order 2] : DOWN
                Slot4WaterTemperature -> Slot4Battery [order 1] : UP
                Slot4WaterTemperature -> Slot4Odometer [order 2] : DOWN
                Slot4Odometer -> Slot4WaterTemperature [order 1] : UP
                Slot4Odometer -> (junction 2938) [order 2] : DOWN
                (junction 2939) -> Slot4Odometer
              2929 -> Slot4FavoritesMenu
              (junction 4243) -> 2930
              Slot4FavoritesMenu -> (junction 4243) [order 1] : EXIT
              (junction 4241) -> 2930 : {favSlot4Sel = currentState;
                  | BLU_FnSaveSlot4Fav(currentState);}
              (junction 3932) -> (junction 4243) [order 2]
              Slot4FavoritesMenu -> (junction 3932) [order 2] : SET
              (junction 3932) -> (junction 4241) [order 1] : [currentState != favSlot1Sel && ...
                  | currentState != favSlot2Sel && ...
                  | currentState != favSlot3Sel ]
            FavoritesSlot1 -> 2879 [order 2] : SET
            2882 -> FavoritesSlot1
            3001 -> FavoritesSlotsMenu
            FavoritesSlot2 -> 2897 [order 1] : SET
            2900 -> FavoritesSlot2
            FavoritesSlotsMenu -> 3004 : EXIT
            FavoritesSlot3 -> 2919 [order 3] : SET
            2922 -> FavoritesSlot3
            FavoritesSlot4 -> 2926 [order 2] : SET
            2927 -> FavoritesSlot4
          state QuickSelectorSubMenu
            state QuickSelectorSubMenu1
              state QuickSelectorUP
                en:
                currentState = eStateName.QUICK_SELECTOR_UP;
              state QuickSelectorDOWN
                en:
                currentState = eStateName.QUICK_SELECTOR_DOWN;
              (default) -> QuickSelectorUP
              QuickSelectorUP -> QuickSelectorDOWN [order 2] : DOWN || UP
              QuickSelectorDOWN -> QuickSelectorUP [order 2] : UP || DOWN
            state QuickSelectorUPSubMenu
              state QS_UP_SubMenu
                (history)
                state QS_UP_RideMode
                  en:
                  currentState = eStateName.QS_UP_RIDE_MODE;
                state QS_UP_ABSMode
                  en:
                  currentState = eStateName.QS_UP_ABS_MODE;
                state QS_UP_MTC
                  en:
                  currentState = eStateName.QS_UP_MTC;
                state QS_UP_TRIP2
                  en:
                  currentState = eStateName.QS_UP_TRIP1;
                state QS_UP_TRIP3
                  en:
                  currentState = eStateName.QS_UP_TRIP2;
                state QS_UP_AUDIO
                  en:
                  currentState = eStateName.QS_UP_AUDIO;
                state QS_UP_NAVIGATION
                  en:
                  currentState = eStateName.QS_UP_NAVIGATION;
                state QS_UP_HEATEDGRIPS
                  en:
                  currentState = eStateName.QS_UP_HEATEDGRIPS;
                state QS_UP_CRUISECONTROL
                  en:
                  currentState = eStateName.QS_UP_CRUISECONTROL;
                state QS_UP_BIKEINFO
                  en:
                  currentState = eStateName.QS_UP_BIKEINFO;
                (default) -> (junction 2806)
                (junction 2806) -> QS_UP_RideMode
                (junction 2808) -> (junction 2806)
                QS_UP_RideMode -> (junction 2812) [order 2] : UP
                (junction 2812) -> (junction 2814)
                QS_UP_RideMode -> QS_UP_ABSMode [order 1] : DOWN
                QS_UP_ABSMode -> QS_UP_RideMode [order 1] : UP
                QS_UP_ABSMode -> QS_UP_MTC [order 2] : DOWN
                QS_UP_MTC -> QS_UP_ABSMode [order 1] : UP
                QS_UP_MTC -> QS_UP_TRIP2 [order 2] : DOWN
                QS_UP_TRIP2 -> QS_UP_MTC [order 1] : UP
                QS_UP_TRIP2 -> QS_UP_TRIP3 [order 2] : DOWN
                QS_UP_TRIP3 -> QS_UP_TRIP2 [order 2] : UP
                (junction 2027) -> QS_UP_TRIP3
                QS_UP_AUDIO -> (junction 2027) [order 2] : UP
                (junction 2021) -> (junction 2027) [order 2]
                QS_UP_TRIP3 -> (junction 1987) [order 1] : DOWN
                (junction 1987) -> QS_UP_AUDIO [order 1] : [CCU_Status == eCCUStatus.installed || ...
                    | CCU_Music_Feature != 0 || ...
                    | CCU_BT_Status != 0]
                (junction 1987) -> (junction 1989) [order 2]
                (junction 2021) -> QS_UP_AUDIO [order 1] : [CCU_Status == eCCUStatus.installed || ...
                    | CCU_Music_Feature != 0 || ...
                    | CCU_BT_Status != 0]
                QS_UP_NAVIGATION -> (junction 2021) [order 2] : UP
                (junction 2018) -> (junction 2021) [order 2]
                QS_UP_AUDIO -> (junction 1989) [order 1] : DOWN
                (junction 1989) -> QS_UP_NAVIGATION [order 1] : [CCU_Status == eCCUStatus.installed || ...
                    | CCU_TbT_Navigation_Feature != 0 || ...
                    | CCU_BT_Status != 0]
                (junction 1989) -> (junction 1995) [order 2]
                (junction 2018) -> QS_UP_NAVIGATION [order 1] : [CCU_Status == eCCUStatus.installed || ...
                    | CCU_TbT_Navigation_Feature != 0 || ...
                    | CCU_BT_Status != 0]
                QS_UP_HEATEDGRIPS -> (junction 2018) [order 2] : UP
                (junction 2015) -> (junction 2018) [order 2]
                QS_UP_NAVIGATION -> (junction 1995) [order 1] : DOWN
                (junction 1995) -> QS_UP_HEATEDGRIPS [order 1] : [Heated_Grips || ...
                    | heatedGrips == eFeatureStatus.available]
                (junction 1995) -> (junction 2000) [order 2]
                (junction 2015) -> QS_UP_HEATEDGRIPS [order 1] : [Heated_Grips || ...
                    | heatedGrips == eFeatureStatus.available]
                QS_UP_CRUISECONTROL -> (junction 2015) [order 2] : UP
                (junction 2012) -> (junction 2015) [order 2]
                QS_UP_HEATEDGRIPS -> (junction 2000) [order 1] : DOWN
                (junction 2000) -> QS_UP_CRUISECONTROL [order 1] : [ECU_SL_Feature !=0]
                (junction 2012) -> QS_UP_CRUISECONTROL [order 1] : [ECU_SL_Feature !=0]
                (junction 2000) -> (junction 2006) [order 2]
                (junction 2010) -> (junction 2012)
                QS_UP_CRUISECONTROL -> (junction 2006) [order 1] : DOWN
                (junction 2814) -> (junction 2006)
                (junction 2006) -> QS_UP_BIKEINFO
                QS_UP_BIKEINFO -> (junction 2010) [order 1] : UP
                QS_UP_BIKEINFO -> (junction 2808) [order 2] : DOWN
              (junction 3952) -> 2817 : {quickSelectorUp = currentState;
                  | BLU_FnSetQuickSelectorUP(quickSelectorUp);}
              QS_UP_SubMenu -> 2817 [order 2] : EXIT
              QS_UP_SubMenu -> (junction 3952) [order 1] : SET
              2804 -> QS_UP_SubMenu
            state QuickSelectorDOWNSubMenu
              state QS_DOWN_SubMenu
                (history)
                state QS_DOWN_RideMode
                  en:
                  currentState = eStateName.QS_DOWN_RIDE_MODE;
                state QS_DOWN_ABSMode
                  en:
                  currentState = eStateName.QS_DOWN_ABS_MODE;
                state QS_DOWN_MTC
                  en:
                  currentState = eStateName.QS_DOWN_MTC;
                state QS_DOWN_TRIP2
                  en:
                  currentState = eStateName.QS_DOWN_TRIP1;
                state QS_DOWN_TRIP3
                  en:
                  currentState = eStateName.QS_DOWN_TRIP2;
                state QS_DOWN_AUDIO
                  en:
                  currentState = eStateName.QS_DOWN_AUDIO;
                state QS_DOWN_NAVIGATION
                  en:
                  currentState = eStateName.QS_DOWN_NAVIGATION;
                state QS_DOWN_HEATEDGRIPS
                  en:
                  currentState = eStateName.QS_DOWN_HEATEDGRIPS;
                state QS_DOWN_CRUISECONTROL
                  en:
                  currentState = eStateName.QS_DOWN_CRUISECONTROL;
                state QS_DOWN_BIKEINFO
                  en:
                  currentState = eStateName.QS_DOWN_BIKEINFO;
                (junction 2821) -> QS_DOWN_RideMode
                (default) -> (junction 2821)
                (junction 2823) -> (junction 2821)
                QS_DOWN_RideMode -> (junction 2826) [order 2] : UP
                (junction 2826) -> (junction 2828)
                QS_DOWN_RideMode -> QS_DOWN_ABSMode [order 1] : DOWN
                QS_DOWN_ABSMode -> QS_DOWN_RideMode [order 1] : UP
                QS_DOWN_ABSMode -> QS_DOWN_MTC [order 2] : DOWN
                QS_DOWN_MTC -> QS_DOWN_ABSMode [order 1] : UP
                QS_DOWN_MTC -> QS_DOWN_TRIP2 [order 2] : DOWN
                QS_DOWN_TRIP2 -> QS_DOWN_MTC [order 1] : UP
                QS_DOWN_TRIP2 -> QS_DOWN_TRIP3 [order 2] : DOWN
                QS_DOWN_TRIP3 -> QS_DOWN_TRIP2 [order 2] : UP
                (junction 2044) -> QS_DOWN_TRIP3
                QS_DOWN_AUDIO -> (junction 2044) [order 2] : UP
                (junction 2046) -> (junction 2044) [order 2]
                QS_DOWN_TRIP3 -> (junction 2045) [order 1] : DOWN
                (junction 2045) -> QS_DOWN_AUDIO [order 1] : [CCU_Status == eCCUStatus.installed || ...
                    | CCU_Music_Feature != 0 || ...
                    | CCU_BT_Status != 0]
                (junction 2045) -> (junction 2047) [order 2]
                (junction 2046) -> QS_DOWN_AUDIO [order 1] : [CCU_Status == eCCUStatus.installed || ...
                    | CCU_Music_Feature != 0 || ...
                    | CCU_BT_Status != 0]
                QS_DOWN_NAVIGATION -> (junction 2046) [order 2] : UP
                (junction 2048) -> (junction 2046) [order 2]
                QS_DOWN_AUDIO -> (junction 2047) [order 1] : DOWN
                (junction 2047) -> QS_DOWN_NAVIGATION [order 1] : [CCU_Status == eCCUStatus.installed || ...
                    | CCU_TbT_Navigation_Feature != 0 || ...
                    | CCU_BT_Status != 0]
                (junction 2047) -> (junction 2049) [order 2]
                (junction 2048) -> QS_DOWN_NAVIGATION [order 1] : [CCU_Status == eCCUStatus.installed || ...
                    | CCU_TbT_Navigation_Feature != 0 || ...
                    | CCU_BT_Status != 0]
                QS_DOWN_HEATEDGRIPS -> (junction 2048) [order 2] : UP
                (junction 2050) -> (junction 2048) [order 2]
                QS_DOWN_NAVIGATION -> (junction 2049) [order 1] : DOWN
                (junction 2049) -> QS_DOWN_HEATEDGRIPS [order 1] : [Heated_Grips || ...
                    | heatedGrips == eFeatureStatus.available]
                (junction 2049) -> (junction 2051) [order 2]
                (junction 2050) -> QS_DOWN_HEATEDGRIPS [order 1] : [Heated_Grips || ...
                    | heatedGrips == eFeatureStatus.available]
                QS_DOWN_CRUISECONTROL -> (junction 2050) [order 2] : UP
                (junction 2052) -> (junction 2050) [order 2]
                QS_DOWN_HEATEDGRIPS -> (junction 2051) [order 1] : DOWN
                (junction 2051) -> QS_DOWN_CRUISECONTROL [order 1] : [ECU_SL_Feature !=0]
                (junction 2052) -> QS_DOWN_CRUISECONTROL [order 1] : [ECU_SL_Feature !=0]
                (junction 2051) -> (junction 2053) [order 2]
                (junction 2054) -> (junction 2052)
                QS_DOWN_CRUISECONTROL -> (junction 2053) [order 1] : DOWN
                (junction 2828) -> (junction 2053)
                (junction 2053) -> QS_DOWN_BIKEINFO
                QS_DOWN_BIKEINFO -> (junction 2054) [order 1] : UP
                QS_DOWN_BIKEINFO -> (junction 2823) [order 2] : DOWN
              (junction 3956) -> 2834
              QS_DOWN_SubMenu -> 2834 [order 2] : EXIT
              QS_DOWN_SubMenu -> (junction 3956) [order 1] : SET
                  | {quickSelectorDown = currentState;
                  | BLU_FnSetQuickSelectorDOWN(quickSelectorDown);}
              2831 -> QS_DOWN_SubMenu
            QuickSelectorUP -> 2805 [order 1] : SET
            2838 -> QuickSelectorSubMenu1
            2818 -> QuickSelectorUP
            QuickSelectorSubMenu1 -> 2842 : EXIT
            QuickSelectorDOWN -> 2832 [order 1] : SET
            2835 -> QuickSelectorDOWN
          state ConnectivityMenu
            state ConnectivitySubMenu
              (history)
              state ConnectivitySubMenu
                state Bluetooth
                  en:
                  currentState = eStateName.CONNECTIVITY_BLUETOOTH;
                state PhonePairing
                  en:
                  currentState = eStateName.CONNECTIVITY_PHONEPAIRING;
                state HeadsetPairing
                  en:
                  currentState = eStateName.CONNECTIVITY_HEADSETPAIRING;
                state HeadsetType
                  en:
                  currentState = eStateName.CONNECTIVITY_HEADSETTYPE;
                (default) -> (junction 2845)
                (junction 2845) -> Bluetooth
                (junction 2853) -> (junction 2845)
                Bluetooth -> (junction 2847) [order 3] : UP
                (junction 2847) -> (junction 2849) : [CCU_BT_Status]
                Bluetooth -> (junction 4012) [order 1] : DOWN
                PhonePairing -> Bluetooth [order 2] : UP
                (junction 4012) -> PhonePairing : [CCU_BT_Status]
                (junction 4070) -> (junction 4012) [order 2]
                PhonePairing -> (junction 4084) [order 1] : DOWN
                (junction 4084) -> (junction 4085)
                HeadsetPairing -> PhonePairing [order 1] : UP
                (junction 4085) -> HeadsetPairing [order 1] : [CCU_Corded_Headset == 0]
                (junction 4085) -> (junction 2849) [order 2]
                (junction 4070) -> HeadsetPairing [order 1] : [CCU_Corded_Headset == 0]
                HeadsetType -> (junction 4070) [order 1] : UP
                HeadsetPairing -> HeadsetType [order 2] : DOWN
                (junction 2849) -> HeadsetType
                HeadsetType -> (junction 2853) [order 3] : DOWN
              state BLUETOOTH_ONOFF
                state BT_Sel
                  state BLUETOOTH_ON
                    en:
                    currentState = eStateName.CONNECTIVITY_BLUETOOTH_ON;
                  state BLUETOOTH_OFF
                    en:
                    currentState = eStateName.CONNECTIVITY_BLUETOOTH_OFF ;
                  (junction 3997) -> BLUETOOTH_ON [order 1] : [CCU_BT_Status]
                  BLUETOOTH_ON -> BLUETOOTH_OFF : DOWN || UP
                  BLUETOOTH_OFF -> BLUETOOTH_ON : DOWN || UP
                  (default) -> (junction 3997)
                  (junction 3997) -> BLUETOOTH_OFF [order 2]
                BT_Sel -> (junction 3666) [order 2] : SET
                (junction 3666) -> 3661 : {BLU_FnConnBTSwitch(currentState);}
                BT_Sel -> 3661 [order 1] : EXIT
                3658 -> (junction 3997)
              state PhoneMenu
                (history)
                state PhonePairinSubMenu
                  state NEW_PAIRING
                    en:
                    currentState = eStateName.PHONE_PAIRING_NEW;
                  state DELETE_PAIRING
                    en:
                    currentState = eStateName.PHONE_PAIRING_DELETE ;
                  (junction 3344) -> NEW_PAIRING [order 2]
                  NEW_PAIRING -> (junction 3972) [order 2] : DOWN || UP
                  NEW_PAIRING -> DELETE_PAIRING [order 3] : [hasChangedTo(btPhonePrngScs,true)]
                  DELETE_PAIRING -> NEW_PAIRING [order 3] : [hasChangedTo(btPhonePrngScs,false)]
                  (junction 3973) -> (junction 3344)
                  (junction 3972) -> (junction 3344)
                  (default) -> (junction 3973)
                  (junction 3344) -> DELETE_PAIRING [order 1] : [btPhonePrngScs]
                  DELETE_PAIRING -> (junction 3972) [order 1] : DOWN || UP
                state PhoneDeviceSearch
                  (history)
                  state BT_PHONE_STRT_SEARCHING
                    en:
                    currentState=eStateName.BT_PHONE_STRT_SEARCHING;
                  state BT_PHONE_FOUND
                    en:
                    currentState=eStateName.BT_PHONE_DVC_LIST;
                  state BT_PHONE_ALREADY_PAIRED
                    en:
                    currentState=eStateName.BT_PHONE_ALREADY_PAIRED;
                  state BT_PHONE_NOT_FOUND [commented out]
                    en:
                    currentState=eStateName.BT_PHONE_NOT_FOUND;
                  state BT_PHONE_PAIRING
                    en:
                    currentState=eStateName.BT_PHONE_PAIRING_INPROGRESS;
                  state BT_PHONE_CHECK_PASSKEY
                    en:
                    currentState=eStateName.BT_PHONE_CHECK_PASSKEY;
                  state BT_PHONE_PAIRING_FAILED [commented out]
                    en:
                    currentState=eStateName.BT_PHONE_PAIRING_FAILED;
                  state BT_PHONE_PAIR_SUCCESS
                    en:
                    currentState=eStateName.BT_PHONE_PAIR_SUCCESS;
                  4016 -> Flow.ButtonTriggeredMenu.Menu.SettingsSubMenu.ConnectivityMenu.ConnectivitySubMenu.PhoneMenu.PhoneDeviceSearch.BT_PHONE_STRT_SEARCHING
                  (default) -> Flow.ButtonTriggeredMenu.Menu.SettingsSubMenu.ConnectivityMenu.ConnectivitySubMenu.PhoneMenu.PhoneDeviceSearch.BT_PHONE_STRT_SEARCHING
                  Flow.ButtonTriggeredMenu.Menu.SettingsSubMenu.ConnectivityMenu.ConnectivitySubMenu.PhoneMenu.PhoneDeviceSearch.BT_PHONE_FOUND -> (junction 3371) [order 1] : UP
                  (junction 3371) -> (junction 3377) : {BLU_FnBTPhoneDvcUp();}
                  Flow.ButtonTriggeredMenu.Menu.SettingsSubMenu.ConnectivityMenu.ConnectivitySubMenu.PhoneMenu.PhoneDeviceSearch.BT_PHONE_STRT_SEARCHING -> Flow.ButtonTriggeredMenu.Menu.SettingsSubMenu.ConnectivityMenu.ConnectivitySubMenu.PhoneMenu.PhoneDeviceSearch.BT_PHONE_FOUND [order 1] : [hasChangedTo(btPhoneFound,true)]
                  (junction 3377) -> Flow.ButtonTriggeredMenu.Menu.SettingsSubMenu.ConnectivityMenu.ConnectivitySubMenu.PhoneMenu.PhoneDeviceSearch.BT_PHONE_FOUND
                  (junction 3375) -> (junction 3377) : {BLU_FnBTPhoneDvcDwn();}
                  Flow.ButtonTriggeredMenu.Menu.SettingsSubMenu.ConnectivityMenu.ConnectivitySubMenu.PhoneMenu.PhoneDeviceSearch.BT_PHONE_STRT_SEARCHING -> (junction 3697) [order 3] : after(BLU_BTSearchDur_Tms,msec)
                  Flow.ButtonTriggeredMenu.Menu.SettingsSubMenu.ConnectivityMenu.ConnectivitySubMenu.PhoneMenu.PhoneDeviceSearch.BT_PHONE_STRT_SEARCHING -> (junction 4173) [order 2] : EXIT
                  Flow.ButtonTriggeredMenu.Menu.SettingsSubMenu.ConnectivityMenu.ConnectivitySubMenu.PhoneMenu.PhoneDeviceSearch.BT_PHONE_FOUND -> (junction 3375) [order 2] : DOWN
                  Flow.ButtonTriggeredMenu.Menu.SettingsSubMenu.ConnectivityMenu.ConnectivitySubMenu.PhoneMenu.PhoneDeviceSearch.BT_PHONE_FOUND -> (junction 3392) [order 3] : EXIT
                  (junction 3697) -> (junction 4173)
                  (junction 4173) -> (junction 3392)
                  Flow.ButtonTriggeredMenu.Menu.SettingsSubMenu.ConnectivityMenu.ConnectivitySubMenu.PhoneMenu.PhoneDeviceSearch.BT_PHONE_FOUND -> (junction 3701) [order 4] : SET
                  (junction 3392) -> (junction 3394)
                  (junction 3701) -> (junction 3705)
                  (junction 3705) -> Flow.ButtonTriggeredMenu.Menu.SettingsSubMenu.ConnectivityMenu.ConnectivitySubMenu.PhoneMenu.PhoneDeviceSearch.BT_PHONE_ALREADY_PAIRED [order 1] : %[phonePaired]
                      | [btPhonePrngScs]
                  (junction 3705) -> (junction 3727) [order 2]
                  Flow.ButtonTriggeredMenu.Menu.SettingsSubMenu.ConnectivityMenu.ConnectivitySubMenu.PhoneMenu.PhoneDeviceSearch.BT_PHONE_NOT_FOUND -> (junction 3394) [commented out] : EXIT
                  Flow.ButtonTriggeredMenu.Menu.SettingsSubMenu.ConnectivityMenu.ConnectivitySubMenu.PhoneMenu.PhoneDeviceSearch.BT_PHONE_ALREADY_PAIRED -> (junction 3394) [order 2] : EXIT
                  (junction 3394) -> (junction 3411)
                  Flow.ButtonTriggeredMenu.Menu.SettingsSubMenu.ConnectivityMenu.ConnectivitySubMenu.PhoneMenu.PhoneDeviceSearch.BT_PHONE_ALREADY_PAIRED -> (junction 3727) [order 1] : SET
                  (junction 3727) -> Flow.ButtonTriggeredMenu.Menu.SettingsSubMenu.ConnectivityMenu.ConnectivitySubMenu.PhoneMenu.PhoneDeviceSearch.BT_PHONE_PAIRING : {BLU_FnBTPhonePairReq();}
                  Flow.ButtonTriggeredMenu.Menu.SettingsSubMenu.ConnectivityMenu.ConnectivitySubMenu.PhoneMenu.PhoneDeviceSearch.BT_PHONE_PAIRING -> Flow.ButtonTriggeredMenu.Menu.SettingsSubMenu.ConnectivityMenu.ConnectivitySubMenu.PhoneMenu.PhoneDeviceSearch.BT_PHONE_CHECK_PASSKEY [order 3] : [hasChangedTo(btPhonePassKeyRcvd,true)]
                  Flow.ButtonTriggeredMenu.Menu.SettingsSubMenu.ConnectivityMenu.ConnectivitySubMenu.PhoneMenu.PhoneDeviceSearch.BT_PHONE_CHECK_PASSKEY -> Flow.ButtonTriggeredMenu.Menu.SettingsSubMenu.ConnectivityMenu.ConnectivitySubMenu.PhoneMenu.PhoneDeviceSearch.BT_PHONE_PAIRING [order 1] : SET
                      | {BLU_FnBTPhonePassKeyChkd();}
                  Flow.ButtonTriggeredMenu.Menu.SettingsSubMenu.ConnectivityMenu.ConnectivitySubMenu.PhoneMenu.PhoneDeviceSearch.BT_PHONE_CHECK_PASSKEY -> (junction 3730) [order 2] : EXIT
                  Flow.ButtonTriggeredMenu.Menu.SettingsSubMenu.ConnectivityMenu.ConnectivitySubMenu.PhoneMenu.PhoneDeviceSearch.BT_PHONE_PAIRING -> (junction 3713) [order 4] : EXIT
                  Flow.ButtonTriggeredMenu.Menu.SettingsSubMenu.ConnectivityMenu.ConnectivitySubMenu.PhoneMenu.PhoneDeviceSearch.BT_PHONE_PAIRING -> (junction 3733) [order 1] : [hasChangedTo(btPhonePairingError,true)]
                  Flow.ButtonTriggeredMenu.Menu.SettingsSubMenu.ConnectivityMenu.ConnectivitySubMenu.PhoneMenu.PhoneDeviceSearch.BT_PHONE_PAIRING -> (junction 3723) [order 2] : [hasChangedTo(btPhonePrngScs,true)]
                  Flow.ButtonTriggeredMenu.Menu.SettingsSubMenu.ConnectivityMenu.ConnectivitySubMenu.PhoneMenu.PhoneDeviceSearch.BT_PHONE_PAIRING_FAILED -> (junction 3411) [commented out] : SET || UP||DOWN || EXIT
                  (junction 3730) -> (junction 3411)
                  (junction 3713) -> (junction 3730)
                  (junction 3733) -> (junction 3713)
                  (junction 3411) -> (junction 3447)
                  Flow.ButtonTriggeredMenu.Menu.SettingsSubMenu.ConnectivityMenu.ConnectivitySubMenu.PhoneMenu.PhoneDeviceSearch.BT_PHONE_PAIR_SUCCESS -> (junction 3447) : after(1,sec)
                  (junction 3447) -> 3390
                  (junction 3723) -> Flow.ButtonTriggeredMenu.Menu.SettingsSubMenu.ConnectivityMenu.ConnectivitySubMenu.PhoneMenu.PhoneDeviceSearch.BT_PHONE_PAIR_SUCCESS : {phonePaired=true;}
                state PhoneBTDvcDelete
                  (history)
                  state BT_PHONE_DEL_PAIRING_WAIT
                    en:
                    currentState=eStateName.BT_PHONE_DEL_PAIRING_WAIT;
                    BLU_FnBTPhoneDvcDel();
                  4019 -> (junction 4091)
                  (junction 4089) -> 3580
                  BT_PHONE_DEL_PAIRING_WAIT -> (junction 4089) [order 1] : EXIT
                  BT_PHONE_DEL_PAIRING_WAIT -> 3580 [order 2] : [hasChangedTo(btPhoneDelErr,true)]
                  (default) -> (junction 4091)
                  (junction 4091) -> BT_PHONE_DEL_PAIRING_WAIT
                  BT_PHONE_DEL_PAIRING_WAIT -> 4093 [order 3] : [hasChangedTo(btPhonePrngScs, false)]
                NEW_PAIRING -> 4017 [order 1] : SET
                3391 -> PhonePairinSubMenu
                (junction 4097) -> NEW_PAIRING
                4094 -> (junction 4097)
                3340 -> (junction 3973)
                DELETE_PAIRING -> 4020 [order 2] : SET
                PhonePairinSubMenu -> 3342 : EXIT
                3569 -> DELETE_PAIRING
              state BT_HeadsetMenu
                state HeadsetPairingSubMenu
                  state HEADSET_PAIRING_NEW
                    en:
                    currentState = eStateName.HEADSET_PAIRING_NEW;
                  state HEADSET_PAIRING_DELETE
                    en:
                    currentState = eStateName.HEADSET_PAIRING_DELETE;
                  (junction 3481) -> HEADSET_PAIRING_NEW [order 2]
                  HEADSET_PAIRING_NEW -> (junction 3967) [order 1] : DOWN || UP
                  HEADSET_PAIRING_NEW -> HEADSET_PAIRING_DELETE [order 3] : [hasChangedTo(btHdstPrngScs,true)]
                  (junction 4137) -> HEADSET_PAIRING_NEW
                  (default) -> (junction 3969)
                  (junction 3969) -> (junction 3481)
                  (junction 3967) -> (junction 3481)
                  (junction 3481) -> HEADSET_PAIRING_DELETE [order 1] : [btHdstPrngScs]
                  HEADSET_PAIRING_DELETE -> (junction 3967) [order 2] : DOWN || UP
                  HEADSET_PAIRING_DELETE -> (junction 4137) [order 1] : [hasChangedTo(btHdstPrngScs,false)]
                state HeadsetDeviceSearch
                  (history)
                  state BT_HEADSET_FOUND
                    en:
                    currentState=eStateName.BT_HEADSET_DVC_LIST;
                  state BT_HEADSET_STRT_SEARCHING
                    en:
                    currentState=eStateName.BT_HEADSET_STRT_SEARCHING;
                  state PhoneDeviceSearch [commented out]
                    state BT_PHONE_STRT_SEARCHING [commented out]
                      en:
                      currentState=eStateName.BT_PHONE_STRT_SEARCHING;
                    state BT_PHONE_FOUND [commented out]
                      en:
                      currentState=eStateName.BT_PHONE_DVC_LIST;
                    state BT_PHONE_ALREADY_PAIRED [commented out]
                      en:
                      currentState=eStateName.BT_PHONE_ALREADY_PAIRED;
                    state BT_PHONE_NOT_FOUND [commented out]
                      en:
                      currentState=eStateName.BT_PHONE_NOT_FOUND;
                    state BT_PHONE_PAIRING [commented out]
                      en:
                      currentState=eStateName.BT_PHONE_PAIRING_INPROGRESS;
                    state BT_PHONE_CHECK_PASSKEY [commented out]
                      en:
                      currentState=eStateName.BT_PHONE_CHECK_PASSKEY;
                    state BT_PHONE_PAIRING_FAILED [commented out]
                      en:
                      currentState=eStateName.BT_PHONE_PAIRING_FAILED;
                    state BT_PHONE_PAIR_SUCCESS [commented out]
                      en:
                      currentState=eStateName.BT_PHONE_PAIR_SUCCESS;
                    (default) -> Flow.ButtonTriggeredMenu.Menu.SettingsSubMenu.ConnectivityMenu.ConnectivitySubMenu.BT_HeadsetMenu.HeadsetDeviceSearch.PhoneDeviceSearch.BT_PHONE_STRT_SEARCHING [commented out]
                    Flow.ButtonTriggeredMenu.Menu.SettingsSubMenu.ConnectivityMenu.ConnectivitySubMenu.BT_HeadsetMenu.HeadsetDeviceSearch.PhoneDeviceSearch.BT_PHONE_FOUND -> (junction 3737) [commented out] : UP
                    (junction 3737) -> (junction 3738) [commented out] : {BLU_FnBTPhoneDvcUp();}
                    Flow.ButtonTriggeredMenu.Menu.SettingsSubMenu.ConnectivityMenu.ConnectivitySubMenu.BT_HeadsetMenu.HeadsetDeviceSearch.PhoneDeviceSearch.BT_PHONE_STRT_SEARCHING -> Flow.ButtonTriggeredMenu.Menu.SettingsSubMenu.ConnectivityMenu.ConnectivitySubMenu.BT_HeadsetMenu.HeadsetDeviceSearch.PhoneDeviceSearch.BT_PHONE_FOUND [commented out] : [hasChangedTo(btPhoneFound,true)]
                    (junction 3738) -> Flow.ButtonTriggeredMenu.Menu.SettingsSubMenu.ConnectivityMenu.ConnectivitySubMenu.BT_HeadsetMenu.HeadsetDeviceSearch.PhoneDeviceSearch.BT_PHONE_FOUND [commented out]
                    (junction 3739) -> (junction 3738) [commented out] : {BLU_FnBTPhoneDvcDwn();}
                    Flow.ButtonTriggeredMenu.Menu.SettingsSubMenu.ConnectivityMenu.ConnectivitySubMenu.BT_HeadsetMenu.HeadsetDeviceSearch.PhoneDeviceSearch.BT_PHONE_STRT_SEARCHING -> (junction 3740) [commented out] : after(BLU_BTSearchDur_Tms,msec)
                    Flow.ButtonTriggeredMenu.Menu.SettingsSubMenu.ConnectivityMenu.ConnectivitySubMenu.BT_HeadsetMenu.HeadsetDeviceSearch.PhoneDeviceSearch.BT_PHONE_FOUND -> (junction 3739) [commented out] : DOWN
                    (junction 3740) -> (junction 3741) [commented out]
                    Flow.ButtonTriggeredMenu.Menu.SettingsSubMenu.ConnectivityMenu.ConnectivitySubMenu.BT_HeadsetMenu.HeadsetDeviceSearch.PhoneDeviceSearch.BT_PHONE_FOUND -> (junction 3741) [commented out] : EXIT
                    Flow.ButtonTriggeredMenu.Menu.SettingsSubMenu.ConnectivityMenu.ConnectivitySubMenu.BT_HeadsetMenu.HeadsetDeviceSearch.PhoneDeviceSearch.BT_PHONE_FOUND -> (junction 3742) [commented out] : SET
                    (junction 3741) -> (junction 3744) [commented out]
                    (junction 3742) -> (junction 3743) [commented out]
                    (junction 3743) -> Flow.ButtonTriggeredMenu.Menu.SettingsSubMenu.ConnectivityMenu.ConnectivitySubMenu.BT_HeadsetMenu.HeadsetDeviceSearch.PhoneDeviceSearch.BT_PHONE_ALREADY_PAIRED [commented out] : [phonePaired]
                    (junction 3743) -> (junction 3745) [commented out]
                    Flow.ButtonTriggeredMenu.Menu.SettingsSubMenu.ConnectivityMenu.ConnectivitySubMenu.BT_HeadsetMenu.HeadsetDeviceSearch.PhoneDeviceSearch.BT_PHONE_NOT_FOUND -> (junction 3744) [commented out] : EXIT
                    Flow.ButtonTriggeredMenu.Menu.SettingsSubMenu.ConnectivityMenu.ConnectivitySubMenu.BT_HeadsetMenu.HeadsetDeviceSearch.PhoneDeviceSearch.BT_PHONE_ALREADY_PAIRED -> (junction 3744) [commented out] : EXIT
                    (junction 3744) -> (junction 3747) [commented out]
                    Flow.ButtonTriggeredMenu.Menu.SettingsSubMenu.ConnectivityMenu.ConnectivitySubMenu.BT_HeadsetMenu.HeadsetDeviceSearch.PhoneDeviceSearch.BT_PHONE_ALREADY_PAIRED -> (junction 3745) [commented out] : SET
                    (junction 3745) -> Flow.ButtonTriggeredMenu.Menu.SettingsSubMenu.ConnectivityMenu.ConnectivitySubMenu.BT_HeadsetMenu.HeadsetDeviceSearch.PhoneDeviceSearch.BT_PHONE_PAIRING [commented out] : {BLU_FnBTPhonePairReq();}
                    Flow.ButtonTriggeredMenu.Menu.SettingsSubMenu.ConnectivityMenu.ConnectivitySubMenu.BT_HeadsetMenu.HeadsetDeviceSearch.PhoneDeviceSearch.BT_PHONE_PAIRING -> Flow.ButtonTriggeredMenu.Menu.SettingsSubMenu.ConnectivityMenu.ConnectivitySubMenu.BT_HeadsetMenu.HeadsetDeviceSearch.PhoneDeviceSearch.BT_PHONE_CHECK_PASSKEY [commented out] : [hasChangedTo(btPhonePassKeyRcvd,true)]
                    Flow.ButtonTriggeredMenu.Menu.SettingsSubMenu.ConnectivityMenu.ConnectivitySubMenu.BT_HeadsetMenu.HeadsetDeviceSearch.PhoneDeviceSearch.BT_PHONE_CHECK_PASSKEY -> Flow.ButtonTriggeredMenu.Menu.SettingsSubMenu.ConnectivityMenu.ConnectivitySubMenu.BT_HeadsetMenu.HeadsetDeviceSearch.PhoneDeviceSearch.BT_PHONE_PAIRING [commented out] : SET
                        | {BLU_FnBTPhonePassKeyChkd();}
                    Flow.ButtonTriggeredMenu.Menu.SettingsSubMenu.ConnectivityMenu.ConnectivitySubMenu.BT_HeadsetMenu.HeadsetDeviceSearch.PhoneDeviceSearch.BT_PHONE_CHECK_PASSKEY -> (junction 3748) [commented out] : EXIT
                    Flow.ButtonTriggeredMenu.Menu.SettingsSubMenu.ConnectivityMenu.ConnectivitySubMenu.BT_HeadsetMenu.HeadsetDeviceSearch.PhoneDeviceSearch.BT_PHONE_PAIRING -> (junction 3746) [commented out] : EXIT
                    Flow.ButtonTriggeredMenu.Menu.SettingsSubMenu.ConnectivityMenu.ConnectivitySubMenu.BT_HeadsetMenu.HeadsetDeviceSearch.PhoneDeviceSearch.BT_PHONE_PAIRING -> (junction 3749) [commented out] : [hasChangedTo(btPhonePairingError,true)]
                    Flow.ButtonTriggeredMenu.Menu.SettingsSubMenu.ConnectivityMenu.ConnectivitySubMenu.BT_HeadsetMenu.HeadsetDeviceSearch.PhoneDeviceSearch.BT_PHONE_PAIRING -> (junction 3750) [commented out] : [hasChangedTo(btPhonePairingScs,true)]
                    Flow.ButtonTriggeredMenu.Menu.SettingsSubMenu.ConnectivityMenu.ConnectivitySubMenu.BT_HeadsetMenu.HeadsetDeviceSearch.PhoneDeviceSearch.BT_PHONE_PAIRING_FAILED -> (junction 3747) [commented out] : SET || UP||DOWN || EXIT
                    (junction 3748) -> (junction 3747) [commented out]
                    (junction 3746) -> (junction 3748) [commented out]
                    (junction 3749) -> (junction 3746) [commented out]
                    (junction 3747) -> (junction 3751) [commented out]
                    (junction 3751) -> 3752 [commented out]
                    Flow.ButtonTriggeredMenu.Menu.SettingsSubMenu.ConnectivityMenu.ConnectivitySubMenu.BT_HeadsetMenu.HeadsetDeviceSearch.PhoneDeviceSearch.BT_PHONE_PAIR_SUCCESS -> (junction 3751) [commented out] : after(3,sec)
                    (junction 3750) -> Flow.ButtonTriggeredMenu.Menu.SettingsSubMenu.ConnectivityMenu.ConnectivitySubMenu.BT_HeadsetMenu.HeadsetDeviceSearch.PhoneDeviceSearch.BT_PHONE_PAIR_SUCCESS [commented out] : {phonePaired=true;}
                  state BT_HEADSET_NOT_FOUND [commented out]
                    en:
                    currentState=eStateName.BT_HEADSET_NOT_FOUND;
                  state BT_HEADSET_ALREADY_PAIRED
                    en:
                    currentState=eStateName.BT_HEADSET_ALREADY_PAIRED;
                  state BT_HEADSET_PAIRING_INPROGRESS
                    en:
                    currentState=eStateName.BT_HEADSET_PAIRING_INPROGRESS;
                  state BT_HEADSET_PAIRING_FAILED
                    en:
                    currentState=eStateName.BT_HEADSET_PAIRING_FAILED;
                  state BT_HEADSET_PAIR_SUCCESS
                    en:
                    currentState=eStateName.BT_HEADSET_PAIR_SUCCESS;
                  4024 -> BT_HEADSET_STRT_SEARCHING
                  (default) -> BT_HEADSET_STRT_SEARCHING
                  BT_HEADSET_FOUND -> (junction 3492) [order 2] : UP
                  (junction 3492) -> (junction 3493) : {BLU_FnBTHeadsetDvcUp();}
                  (junction 3493) -> BT_HEADSET_FOUND
                  BT_HEADSET_STRT_SEARCHING -> BT_HEADSET_FOUND [order 1] : [hasChangedTo(btHeadsetFound,true)]
                      | {headsetPaired = btHdstPrngScs;}
                  (junction 3495) -> (junction 3493) : {BLU_FnBTHeadsetDvcDwn();}
                  BT_HEADSET_STRT_SEARCHING -> (junction 3494) [order 3] : after(BLU_BTSearchDur_Tms,msec)
                  BT_HEADSET_FOUND -> (junction 3494) [order 4] : EXIT
                  BT_HEADSET_FOUND -> (junction 3495) [order 3] : DOWN
                  (junction 3494) -> (junction 4180)
                  BT_HEADSET_STRT_SEARCHING -> (junction 4178) [order 2] : EXIT
                  BT_HEADSET_FOUND -> (junction 3795) [order 1] : SET
                  (junction 3795) -> (junction 3796)
                  (junction 4178) -> (junction 4180)
                  (junction 4180) -> (junction 3496)
                  (junction 3796) -> BT_HEADSET_ALREADY_PAIRED [order 1] : [headsetPaired]
                  (junction 3796) -> (junction 3800) [order 2]
                  BT_HEADSET_NOT_FOUND -> (junction 3496) [commented out] : EXIT
                  BT_HEADSET_ALREADY_PAIRED -> (junction 3496) [order 1] : EXIT
                  (junction 3496) -> (junction 3498)
                  BT_HEADSET_ALREADY_PAIRED -> (junction 3800) [order 2] : SET
                  (junction 3800) -> BT_HEADSET_PAIRING_INPROGRESS : {BLU_FnBTHeadsetPairReq();}
                  BT_HEADSET_PAIRING_INPROGRESS -> BT_HEADSET_PAIRING_FAILED [order 2] : [hasChangedTo(btHeadsetPairingError,true)]
                  BT_HEADSET_PAIRING_FAILED -> (junction 3498) : SET || UP||DOWN || EXIT
                  (junction 3498) -> (junction 3500)
                  BT_HEADSET_PAIRING_INPROGRESS -> (junction 3803) [order 1]
                  BT_HEADSET_PAIRING_INPROGRESS -> (junction 3805) [order 3] : EXIT
                  (junction 3500) -> 3501
                  BT_HEADSET_PAIR_SUCCESS -> (junction 3500) : after(3,sec)
                      | {headsetPaired = btHdstPrngScs;}
                  (junction 3803) -> BT_HEADSET_PAIR_SUCCESS : [hasChangedTo(btHdstPrngScs,true)]
                  (junction 3807) -> (junction 3500)
                  (junction 3805) -> (junction 3807)
                state HeadsetBTDvcDelete
                  (history)
                  state BT_HEADSET_DEL_PAIRING_WAIT
                    en:
                    currentState=eStateName.BT_HEADSET_DEL_PAIRING_WAIT;
                    BLU_FnBTHeadsetDvcDel();
                  (junction 4127) -> 3632
                  4027 -> (junction 4126)
                  BT_HEADSET_DEL_PAIRING_WAIT -> (junction 4127) [order 1] : EXIT
                  BT_HEADSET_DEL_PAIRING_WAIT -> 3632 [order 2] : [hasChangedTo(btHdstDelErr,true)]
                      | {headsetPaired = btHdstPrngScs;}
                  (default) -> (junction 4126)
                  (junction 4126) -> BT_HEADSET_DEL_PAIRING_WAIT
                  BT_HEADSET_DEL_PAIRING_WAIT -> 4118 [order 3] : [hasChangedTo(btHdstPrngScs,false)]
                HEADSET_PAIRING_NEW -> 4025 [order 2] : SET
                3470 -> HeadsetPairingSubMenu
                3471 -> (junction 3969)
                (junction 4134) -> (junction 4137)
                4131 -> (junction 4134)
                HeadsetPairingSubMenu -> 3472 : EXIT
                HEADSET_PAIRING_DELETE -> 4028 [order 3] : SET
                3629 -> HEADSET_PAIRING_DELETE
              state HeadsetTypeMenu
                state HeadsetSel
                  (history)
                  state HEADSET_CORDED
                    en:
                    currentState = eStateName.HEADSETTYPE_CORDED;
                  state HEADSET_BLUETOOTH
                    en:
                    currentState = eStateName.HEADSETTYPE_BLUETOOTH ;
                  (junction 4073) -> HEADSET_CORDED [order 1] : [CCU_Corded_Headset == 1]
                  (junction 4073) -> (junction 4075) [order 2]
                  HEADSET_CORDED -> HEADSET_BLUETOOTH [order 1] : DOWN || UP
                  HEADSET_BLUETOOTH -> HEADSET_CORDED [order 1] : DOWN || UP
                  (junction 4075) -> HEADSET_BLUETOOTH
                3645 -> (junction 4073)
                HEADSET_CORDED -> (junction 4081) [order 2] : SET
                (junction 4081) -> 3648 : {BLU_FnHdstSelCord();}
                HeadsetSel -> 3648 : EXIT
                (junction 3653) -> 3648 : {BLU_FnHdstSelBT();}
                HEADSET_BLUETOOTH -> (junction 3653) [order 2] : SET
              Bluetooth -> 3659 [order 2] : SET
              3662 -> Bluetooth
              (default) -> Flow.ButtonTriggeredMenu.Menu.SettingsSubMenu.ConnectivityMenu.ConnectivitySubMenu.ConnectivitySubMenu
              PhonePairing -> 3461 [order 3] : SET
              3343 -> PhonePairing
              HeadsetPairing -> 3467 [order 3] : SET
              3466 -> HeadsetPairing
              HeadsetType -> 3646 [order 2] : SET
              3649 -> HeadsetType
            state AppReqMenu
              en:
              popUpState = eStateName.POPUP_REG_APP_REPLY;
            state CnfrmAppReqWait
            2856 -> (junction 2845)
            Flow.ButtonTriggeredMenu.Menu.SettingsSubMenu.ConnectivityMenu.ConnectivitySubMenu.ConnectivitySubMenu -> 2859 : EXIT
            Flow.ButtonTriggeredMenu.Menu.SettingsSubMenu.ConnectivityMenu.ConnectivitySubMenu -> AppReqMenu : [hasChangedTo(rgstrAppReply,0)]
            CnfrmAppReqWait -> Flow.ButtonTriggeredMenu.Menu.SettingsSubMenu.ConnectivityMenu.ConnectivitySubMenu : after(1,sec)
            AppReqMenu -> (junction 3988) [order 1] : SET
                | {cnfrmAppReg = 0;}
            (junction 3988) -> CnfrmAppReqWait : {BLU_FnCnctvtyCnfrmAppReg(cnfrmAppReg);}
            (junction 3993) -> (junction 3988)
            AppReqMenu -> (junction 3993) [order 2] : EXIT
                | {cnfrmAppReg = 15}
          state QuickShifterMenu
            state QuickShifterSubMenu
              (history)
              state QuickShifterOFF
                en:
                currentState = eStateName.QUICKSHIFTER_OFF;
              state QuickShifterON
                en:
                currentState = eStateName.QUICKSHIFTER_ON;
              (default) -> QuickShifterOFF
              QuickShifterOFF -> QuickShifterON : DOWN || UP
              QuickShifterON -> QuickShifterOFF : UP || DOWN
            2785 -> QuickShifterSubMenu
            QuickShifterSubMenu -> (junction 3912) [order 2] : SET
                | {BLU_FnQuickShifterSwitch(currentState);}
            (junction 3912) -> 2790
            QuickShifterSubMenu -> 2790 [order 1] : EXIT
          state ShiftLightSubMenu
            state OdoLessKm
              en:
              currentState = eStateName.ODO_MSG_KM;
            state ShiftLightMenu1
              (history)
              state SL_RPM1
                en:
                currentState = eStateName.SL_RPM1;
              state SL_RPM2
                en:
                currentState = eStateName.SL_RPM2;
              state ShiftLight
                en:
                currentState = eStateName.SHIFT_LIGHT_ON_OFF;
              SL_RPM1 -> (junction 2774) [order 2]
              (junction 2774) -> (junction 2776) [order 2] : UP
              SL_RPM1 -> SL_RPM2 [order 1] : DOWN
              SL_RPM2 -> SL_RPM1 [order 2] : UP
              SL_RPM2 -> Flow.ButtonTriggeredMenu.Menu.SettingsSubMenu.ShiftLightSubMenu.ShiftLightMenu1.ShiftLight [order 3] : DOWN
              Flow.ButtonTriggeredMenu.Menu.SettingsSubMenu.ShiftLightSubMenu.ShiftLightMenu1.ShiftLight -> SL_RPM2 [order 1] : UP
              (junction 2776) -> Flow.ButtonTriggeredMenu.Menu.SettingsSubMenu.ShiftLightSubMenu.ShiftLightMenu1.ShiftLight
            state RPM1menu
              state RPM1menu1
                en:
                currentState = eStateName.SL_SET_RPM1;
              3902 -> (junction 3156)
              (default) -> (junction 3156)
              (junction 3156) -> (junction 3162) [order 1] : [rpm1 >= 5000]
              (junction 3156) -> (junction 3159) [order 2]
              (junction 3162) -> Flow.ButtonTriggeredMenu.Menu.SettingsSubMenu.ShiftLightSubMenu.RPM1menu.RPM1menu1
              (junction 3159) -> Flow.ButtonTriggeredMenu.Menu.SettingsSubMenu.ShiftLightSubMenu.RPM1menu.RPM1menu1 : {rpm1=5000;}
              Flow.ButtonTriggeredMenu.Menu.SettingsSubMenu.ShiftLightSubMenu.RPM1menu.RPM1menu1 -> (junction 1911) [order 1] : UP
              (junction 1911) -> (junction 3165) [order 1] : [rpm1<11000 && rpm1 >= 5000]
              (junction 1911) -> (junction 1913) [order 2]
              (junction 3165) -> (junction 3167) : {rpm1 = rpm1+100;}
              Flow.ButtonTriggeredMenu.Menu.SettingsSubMenu.ShiftLightSubMenu.RPM1menu.RPM1menu1 -> (junction 1921) [order 3] : SET || EXIT
              (junction 1921) -> (junction 1925) [order 2]
              (junction 1921) -> (junction 1923) [order 1] : [rpm1 > rpm2]
              (junction 1913) -> Flow.ButtonTriggeredMenu.Menu.SettingsSubMenu.ShiftLightSubMenu.RPM1menu.RPM1menu1
              (junction 3167) -> (junction 1913)
              (junction 1914) -> (junction 1913) [order 2]
              (junction 3170) -> (junction 3167) : {rpm1 = rpm1-100;}
              (junction 1923) -> (junction 1925) : {rpm2 = rpm1;}
              (junction 1925) -> 3899
              Flow.ButtonTriggeredMenu.Menu.SettingsSubMenu.ShiftLightSubMenu.RPM1menu.RPM1menu1 -> (junction 1914) [order 2] : DOWN
              (junction 1914) -> (junction 3170) [order 1] : [rpm1>5000 && rpm1 <= 11000]
            state RPM2menu
              state RPM1menu1
                en:
                currentState = eStateName.SL_SET_RPM2;
              (junction 3173) -> (junction 3174) [order 1] : [rpm2>=5000]
              3894 -> (junction 3173)
              (default) -> (junction 3173)
              (junction 3173) -> (junction 3177) [order 2]
              (junction 3174) -> Flow.ButtonTriggeredMenu.Menu.SettingsSubMenu.ShiftLightSubMenu.RPM2menu.RPM1menu1
              (junction 3177) -> Flow.ButtonTriggeredMenu.Menu.SettingsSubMenu.ShiftLightSubMenu.RPM2menu.RPM1menu1 : {rpm2 = 5000;}
              Flow.ButtonTriggeredMenu.Menu.SettingsSubMenu.ShiftLightSubMenu.RPM2menu.RPM1menu1 -> (junction 1903) [order 1] : UP
              (junction 1903) -> (junction 3184) [order 1] : [rpm2 >=5000 && rpm2<11000]
              (junction 1903) -> (junction 1905) [order 2]
              (junction 3184) -> (junction 3182) : {rpm2 = rpm2+100;}
              Flow.ButtonTriggeredMenu.Menu.SettingsSubMenu.ShiftLightSubMenu.RPM2menu.RPM1menu1 -> (junction 1931) [order 3] : SET || EXIT
              (junction 1931) -> (junction 1935) [order 2]
              (junction 1931) -> (junction 1933) [order 1] : [ rpm2 < rpm1]
              (junction 3182) -> (junction 1905)
              (junction 1905) -> Flow.ButtonTriggeredMenu.Menu.SettingsSubMenu.ShiftLightSubMenu.RPM2menu.RPM1menu1
              (junction 3180) -> (junction 3182) : {rpm2 = rpm2-100;}
              (junction 1907) -> (junction 1905) [order 2]
              (junction 1933) -> (junction 1935) : {rpm1 = rpm2;}
              (junction 1935) -> 3890
              Flow.ButtonTriggeredMenu.Menu.SettingsSubMenu.ShiftLightSubMenu.RPM2menu.RPM1menu1 -> (junction 1907) [order 2] : DOWN
              (junction 1907) -> (junction 3180) [order 1] : [rpm2 >5000 && rpm2<=11000]
            state ShiftLightSubMenu
              state ShiftLightOnOffMenu
                (history)
                state ShiftLightON
                  en:
                  currentState = eStateName.SHIFT_LIGHT_ON;
                state ShiftLightOFF
                  en:
                  currentState = eStateName.SHIFT_LIGHT_OFF;
                ShiftLightON -> ShiftLightOFF [order 1] : DOWN || UP
                ShiftLightOFF -> ShiftLightON [order 1] : UP || DOWN
              3886 -> ShiftLightON
              ShiftLightON -> (junction 1868) [order 2] : SET
              (junction 1868) -> (junction 1870) : {BLU_FnShiftLightON();
                  | ShiftLightStatus = 1;}
              ShiftLightOnOffMenu -> (junction 1870) : EXIT
              (junction 1870) -> 3884
              (junction 1871) -> (junction 1870) : {BLU_FnShiftLightOFF();
                  | ShiftLightStatus = 0;}
              ShiftLightOFF -> (junction 1871) [order 2] : SET
            state OdoLessMiles
              en:
              currentState = eStateName.ODO_MSG_MILES;
            (junction 3906) -> (junction 3907)
            (junction 3907) -> 2782
            ShiftLightMenu1 -> (junction 3906) : EXIT
            (junction 2774) -> (junction 1884) [order 1] : SET
            (junction 1884) -> 3903 : [ShiftLightStatus == 1]
            (junction 1835) -> SL_RPM1
            OdoLessKm -> (junction 1854) : [after(5,sec)]
            (junction 1838) -> OdoLessKm [order 2]
            (junction 1844) -> (junction 1835)
            3900 -> ShiftLightMenu1
            2779 -> (junction 1832)
            (junction 1832) -> (junction 1838) [order 1] : [odoUnits == 0]
            (junction 1838) -> (junction 1844) [order 1] : [odoValue > 1000]
            (junction 1842) -> (junction 1844)
            (junction 1832) -> (junction 1848) [order 2]
            (junction 1897) -> 3895 : [ShiftLightStatus == 1]
            SL_RPM2 -> (junction 1897) [order 1] : SET
            (junction 1854) -> 2782
            OdoLessMiles -> (junction 1854) : [after(5,sec)]
            3891 -> ShiftLightMenu1
            (junction 1848) -> (junction 1842) [order 1] : [odoValue > 600]
            (junction 1848) -> OdoLessMiles [order 2]
            (junction 2771) -> (junction 1842)
            Flow.ButtonTriggeredMenu.Menu.SettingsSubMenu.ShiftLightSubMenu.ShiftLightMenu1.ShiftLight -> 3887 [order 2] : SET
            Flow.ButtonTriggeredMenu.Menu.SettingsSubMenu.ShiftLightSubMenu.ShiftLightMenu1.ShiftLight -> (junction 2771) [order 3] : DOWN
            3885 -> ShiftLightMenu1
          state ClockSubMenu
            state ClockDateMenu
              (history)
              state Time
                en:
                currentState = eStateName.CLOCK_TIME;
              state Date
                en:
                currentState = eStateName.CLOCK_DATE;
              state ClockFormat
                en:
                currentState = eStateName.CLOCK_CLOCK_FORMAT;
              state DateFormat
                en:
                currentState = eStateName.CLOCK_DATE_FORMAT;
              (junction 2748) -> Time
              Time -> (junction 2753) [order 2]
              (junction 2749) -> (junction 2748)
              (junction 2753) -> (junction 2755) [order 2] : UP
              Time -> Date [order 1] : DOWN
              Date -> Time [order 1] : UP
              Date -> ClockFormat [order 2] : DOWN
              ClockFormat -> Date [order 2] : UP
              ClockFormat -> DateFormat [order 1] : DOWN
              DateFormat -> ClockFormat [order 1] : UP
              (junction 2755) -> DateFormat
              DateFormat -> (junction 2749) [order 2] : DOWN
            state TimeSubMenu
              state TimeHours
                en:
                currentState = eStateName.TIME_HOURS;
              state TimeMinutes
                en:
                currentState = eStateName.TIME_MINUTES;
              TimeHours -> (junction 3423) [order 5] : longUP
                  | {jumpDigits = 5;}
              (junction 3423) -> (junction 881)
              TimeHours -> (junction 881) [order 3] : UP
                  | {jumpDigits=1;}
              (junction 881) -> (junction 883) : {BLU_FnClkIncHrs(jumpDigits);}
              (junction 883) -> TimeHours
              (junction 888) -> (junction 883) : {BLU_FnClkDecHrs(jumpDigits);}
              2765 -> TimeHours
              TimeHours -> (junction 888) [order 4] : DOWN
                  | {jumpDigits=1;}
              (junction 3428) -> (junction 888)
              TimeHours -> (junction 3428) [order 6] : longDOWN
                  | {jumpDigits=5;}
              TimeHours -> (junction 875) [order 2] : EXIT
              TimeHours -> TimeMinutes [order 1] : SET
              TimeMinutes -> TimeHours [order 1] : EXIT
              (junction 875) -> 2763
              TimeMinutes -> (junction 875) [order 2] : SET
                  | {BLU_FnClkSaveTime();}
              TimeMinutes -> (junction 3438) [order 6] : longUP
                  | {jumpDigits=5;}
              (junction 3438) -> (junction 895)
              TimeMinutes -> (junction 895) [order 3] : UP
                  | {jumpDigits=1;}
              (junction 895) -> (junction 898) : {BLU_FnClkIncMins(jumpDigits);}
              (junction 898) -> TimeMinutes
              (junction 903) -> (junction 898) : {BLU_FnClkDecMins(jumpDigits);}
              TimeMinutes -> (junction 903) [order 4] : DOWN
                  | {jumpDigits=1;}
              (junction 3433) -> (junction 903)
              TimeMinutes -> (junction 3433) [order 5] : longDOWN
                  | {jumpDigits=5;}
            state DateSubMenu
              state DateDigit1
                en:
                currentState = eStateName.CLOCK_FORMAT_DIGIT_1;
              state DateDigit2
                en:
                currentState = eStateName.CLOCK_FORMAT_DIGIT_2;
              state DateDigit3
                en:
                currentState = eStateName.CLOCK_FORMAT_DIGIT_3;
              DateDigit1 -> (junction 909) [order 3] : UP
              (junction 909) -> (junction 910) : {BLU_FnClkIncDateDig1();}
              3322 -> DateDigit1
              (junction 910) -> DateDigit1
              (junction 911) -> (junction 910) : {BLU_FnClkDecDateDig1();}
              DateDigit1 -> (junction 912) [order 2] : EXIT
              DateDigit1 -> (junction 911) [order 4] : DOWN
              (junction 912) -> (junction 948)
              DateDigit1 -> DateDigit2 [order 1] : SET
              DateDigit2 -> DateDigit1 [order 1] : EXIT
              DateDigit2 -> (junction 913) [order 2] : UP
              (junction 913) -> (junction 914) : {BLU_FnClkIncDateDig2();}
              (junction 914) -> DateDigit2
              (junction 915) -> (junction 914) : {BLU_FnClkDecDateDig2();}
              (junction 948) -> 3325
              (junction 952) -> (junction 948) : {BLU_FnClkSaveDate();}
              DateDigit2 -> (junction 915) [order 3] : DOWN
              DateDigit2 -> DateDigit3 [order 4] : SET
              DateDigit3 -> DateDigit2 [order 3] : EXIT
              DateDigit3 -> (junction 938) [order 1] : UP
              (junction 938) -> (junction 939) : {BLU_FnClkIncDateDig3();}
              DateDigit3 -> (junction 952) [order 4] : SET
              (junction 939) -> DateDigit3
              (junction 940) -> (junction 939) : {BLU_FnClkDecDateDig3();}
              DateDigit3 -> (junction 940) [order 2] : DOWN
            state SetClockFormat
              (history)
              state SetClockFormatMenu
                state Clock12H
                  en:
                  currentState = eStateName.CLOCK_FORMAT_12H;
                state Clock24H
                  en:
                  currentState = eStateName.CLOCK_FORMAT_24H;
                Clock12H -> Clock24H : UP || DOWN
                Clock24H -> Clock12H : UP || DOWN
              3278 -> Clock12H
              SetClockFormatMenu -> 3286 [order 1] : EXIT
              (junction 3675) -> 3286
              SetClockFormatMenu -> (junction 3675) [order 2] : SET
                  | {BLU_FnClkFrmtTgle(currentState);}
            state SetDateFormat
              state SetDateFormatMenu
                (history)
                state DateFormat1
                  en:
                  currentState = eStateName.DATE_FORMAT_DDMMYYYY;
                state DateFormat2
                  en:
                  currentState = eStateName.DATE_FORMAT_MMDDYYYY;
                state DateFormat3
                  en:
                  currentState = eStateName.DATE_FORMAT_YYYYMMDD;
                (default) -> DateFormat1
                (junction 3293) -> DateFormat1
                DateFormat1 -> (junction 3311) [order 2] : UP
                (junction 3294) -> (junction 3293)
                (junction 3311) -> (junction 3313)
                DateFormat2 -> DateFormat1 [order 2] : UP
                DateFormat1 -> DateFormat2 [order 1] : DOWN
                DateFormat3 -> DateFormat2 [order 2] : UP
                DateFormat2 -> DateFormat3 [order 1] : DOWN
                DateFormat3 -> (junction 3294) [order 1] : DOWN
                (junction 3313) -> DateFormat3
              3304 -> DateFormat1
              SetDateFormatMenu -> 3318 [order 1] : EXIT
              (junction 3672) -> 3318 : {BLU_FnDateFrmtTgle(currentState);}
              SetDateFormatMenu -> (junction 3672) [order 2] : SET
            2758 -> (junction 2748)
            (junction 2753) -> 2766 [order 1] : SET
            2764 -> (junction 3678)
            (junction 3678) -> (junction 3680)
            ClockDateMenu -> 2761 : EXIT
            Date -> 3323 [order 3] : SET
            3326 -> (junction 3680)
            (junction 3680) -> (junction 3683)
            ClockFormat -> 3279 [order 3] : SET
            3287 -> (junction 3683)
            (junction 3683) -> (junction 3686)
            DateFormat -> 3305 [order 3] : SET
            (junction 3686) -> ClockDateMenu
            3319 -> (junction 3686)
          state UnitsSubMenu
            state UnitsMenu
              (history)
              state Distance
                en:
                currentState = eStateName.DISTANCE;
              state Temperature
                en:
                currentState = eStateName.TEMPERATURE;
              state Consumption
                en:
                currentState = eStateName.CONSUMPTION;
              (junction 2717) -> Distance
              (junction 2719) -> (junction 2717)
              Distance -> (junction 2724) [order 3] : UP
              (junction 2724) -> (junction 2726)
              Distance -> Temperature [order 1] : DOWN
              Temperature -> Distance [order 1] : UP
              Temperature -> Consumption [order 2] : DOWN
              Consumption -> Temperature [order 1] : UP
              (junction 2726) -> Consumption
              Consumption -> (junction 2719) [order 3] : DOWN
            state DistanceSubMenu
              state DstnceMenu
                (history)
                state Kilometer
                  en:
                  currentState = eStateName.DISTANCE_KILOMETER;
                state Miles
                  en:
                  currentState = eStateName.DISTANCE_MILES;
                Kilometer -> Miles : DOWN || UP
                Miles -> Kilometer : UP || DOWN
              3846 -> Kilometer
              DstnceMenu -> 3849 [order 1] : EXIT
              (junction 3854) -> 3849 : {BLU_FnSETDistUnits(currentState);}
              DstnceMenu -> (junction 3854) [order 2] : SET
            state TemperatureSubMenu
              state TempUnitsMenu
                (history)
                state Celsius
                  en:
                  currentState = eStateName.TEMPERATURE_CELSIUS;
                state Farenheit
                  en:
                  currentState = eStateName.TEMPERATURE_FARENHEIT;
                Celsius -> Farenheit : DOWN || UP
                Farenheit -> Celsius : UP || DOWN
              3859 -> Celsius
              TempUnitsMenu -> (junction 3867) [order 2] : SET
              (junction 3867) -> 3862 : {BLU_FnSETTempUnits(currentState);}
              TempUnitsMenu -> 3862 [order 1] : EXIT
            state ConsumptionSubMenu
              state ConsUnits
                (history)
                state litres_100km
                  en:
                  currentState = eStateName.CONSUMPTION_LTR_PER_100KM;
                state km_l
                  en:
                  currentState = eStateName.CONSUMPTION_KM_PER_LTR;
                state USg_100mile
                  en:
                  currentState = eStateName.CONSUMPTION_USG_PER_100MI;
                state Mi_USg
                  en:
                  currentState = eStateName.CONSUMPTION_MI_PER_USG;
                state Mi_Litre
                  en:
                  currentState = eStateName.CONSUMPTION_MI_PER_LTR;
                state UKg_100Mi
                  en:
                  currentState = eStateName.CONSUMPTION_UKG_PER_100MI;
                state Mi_UKg
                  en:
                  currentState = eStateName.CONSUMPTION_MI_PER_UKG;
                state Li_100Mi
                  en:
                  currentState = eStateName.CONSUMPTION_L_PER_100MI;
                (default) -> (junction 2738)
                litres_100km -> (junction 2742) [order 2] : UP
                (junction 2738) -> litres_100km
                (junction 2742) -> (junction 2744)
                (junction 2737) -> (junction 2738)
                litres_100km -> km_l [order 1] : DOWN
                km_l -> litres_100km [order 1] : UP
                km_l -> USg_100mile [order 2] : DOWN
                USg_100mile -> km_l [order 1] : UP
                USg_100mile -> Mi_USg [order 2] : DOWN
                Mi_USg -> USg_100mile [order 1] : UP
                Mi_USg -> Mi_Litre [order 2] : DOWN
                Mi_Litre -> Mi_USg [order 1] : UP
                Mi_Litre -> UKg_100Mi [order 2] : DOWN
                UKg_100Mi -> Mi_Litre [order 1] : UP
                UKg_100Mi -> Mi_UKg [order 2] : DOWN
                Mi_UKg -> UKg_100Mi [order 1] : UP
                Mi_UKg -> Li_100Mi [order 2] : DOWN
                Li_100Mi -> Mi_UKg [order 1] : UP
                Li_100Mi -> (junction 2737) [order 2] : DOWN
                (junction 2744) -> Li_100Mi
              3872 -> (junction 2738)
              ConsUnits -> 3875 [order 1] : EXIT
              (junction 3880) -> 3875 : {BLU_FnSETConsUnits(currentState);}
              ConsUnits -> (junction 3880) [order 2] : SET
            (default) -> UnitsMenu
            2729 -> (junction 2717)
            Distance -> 3847 [order 2] : SET
            3850 -> UnitsMenu
            UnitsMenu -> 2732 : EXIT
            Temperature -> 3860 [order 3] : SET
            3863 -> UnitsMenu
            Consumption -> 3873 [order 2] : SET
            3876 -> UnitsMenu
          state LanguageSubMenu
            state LanguageSetSubMenu
              (history)
              state EnglishUS
                en:
                currentState = eStateName.ENGLISH_US;
              state EnglishUK
                en:
                currentState = eStateName.ENGLISH_UK;
              state German
                en:
                currentState = eStateName.GERMAN;
              state Italian
                en:
                currentState = eStateName.ITALIAN;
              state French
                en:
                currentState = eStateName.FRENCH;
              state Spanish
                en:
                currentState = eStateName.SPANISH;
              (junction 2684) -> EnglishUS
              (junction 2681) -> (junction 2684)
              EnglishUS -> (junction 2688) [order 2] : UP
              (junction 2688) -> (junction 2690)
              EnglishUS -> EnglishUK [order 1] : DOWN
              EnglishUK -> EnglishUS [order 1] : UP
              EnglishUK -> German [order 2] : DOWN
              German -> EnglishUK [order 1] : UP
              German -> Italian [order 2] : DOWN
              Italian -> German [order 1] : UP
              Italian -> French [order 2] : DOWN
              French -> Italian [order 1] : UP
              French -> Spanish [order 2] : DOWN
              Spanish -> French [order 1] : UP
              (junction 2690) -> Spanish
              Spanish -> (junction 2681) [order 2] : DOWN
            2676 -> (junction 2684)
            LanguageSetSubMenu -> 2694 [order 1] : EXIT
            (junction 3840) -> 2694 : {BLU_FnSETLanguage(currentState);}
            LanguageSetSubMenu -> (junction 3840) [order 2] : SET
          state HeatingGripsSettingsSubMenu
            state HtdGripsSel
              (history)
              state HeatingGripsNotAvailable
                en:
                currentState = eStateName.HEATING_GRIPS_NOT_AVAILABLE;
              state HeatingGripsAvailable
                en:
                currentState = eStateName.HEATING_GRIPS_AVAILABLE;
              HeatingGripsNotAvailable -> HeatingGripsAvailable [order 1] : DOWN || UP
              HeatingGripsAvailable -> HeatingGripsNotAvailable [order 1] : DOWN || UP
              HeatingGripsAvailable -> HeatingGripsAvailable [commented out] : SET
                  | {heatedGrips = eFeatureStatus.available;
                  | BLU_FnSetHeatedGrips(heatedGrips);}
                  | //TBD Heated_Grips variable set
            state HCU_GripHeat_LvlChk
              en:
              currentState = eStateName.HCU_GRIP_HEAT_LVL_CHK;
            HeatingGripsNotAvailable -> 3836 [order 2] : SET
                | {heatedGrips = eFeatureStatus.notAvailable;
                | DASH_Grip_Installation = 0;
                | BLU_FnSetHeatedGrips(heatedGrips);}
                | //TBD Heated_Grips variable set
            (junction 3822) -> 3836
            3832 -> HeatingGripsNotAvailable
            HtdGripsSel -> (junction 3822) : EXIT
            (junction 3828) -> (junction 3822) : [HCU_Grip_Heat_Level_Res ==0 || after(3,sec)]
            HCU_GripHeat_LvlChk -> (junction 3822) [order 1] : [HCU_Grip_Heat_Level_Res !=0]
                | {heatedGrips = eFeatureStatus.notAvailable;}
            HCU_GripHeat_LvlChk -> (junction 3828) [order 2]
            HeatingGripsAvailable -> HCU_GripHeat_LvlChk [order 2] : SET
                | {heatedGrips = eFeatureStatus.available;
                | DASH_Grip_Installation = 1;}
                | //TBD Heated_Grips variable set
          state ExtraFunctionsSubMenu
            en:
            currentState = eStateName.EXTRA_FUNCTIONS_SUB_MN;
          Favourites -> 3002 [order 1] : SET
          2698 -> (junction 2702)
          3005 -> (junction 2513)
          (junction 2513) -> (junction 2515)
          SettingsMenuScreens -> 2714 : EXIT
          QuickSelector -> 2839 [order 1] : SET
          2843 -> (junction 2515)
          (junction 2515) -> (junction 2517)
          (junction 1102) -> 2857 [order 1] : SET
          2860 -> (junction 2517)
          (junction 2517) -> (junction 2519)
          (junction 1134) -> 2786 [order 2] : SET
          2791 -> (junction 2519)
          (junction 2519) -> (junction 2521)
          Flow.ButtonTriggeredMenu.Menu.SettingsSubMenu.SettingsMenuScreens.ShiftLight -> 2780 [order 3] : SET
          2783 -> (junction 2521)
          (junction 2521) -> (junction 2523)
          4263 -> (junction 4277)
          (junction 4277) -> 2759
          (junction 715) -> (junction 4277) [order 2] : SET
          2762 -> (junction 2523)
          (junction 2523) -> (junction 2525)
          Units -> 2730 [order 3] : SET
          2733 -> (junction 2525)
          (junction 2525) -> (junction 2527)
          Language -> 2677 [order 3] : SET
          2695 -> (junction 2527)
          (junction 2527) -> (junction 2529)
          HeatedGripsSettingsMenu -> 3833 [order 3] : SET
          3837 -> (junction 2529)
          (junction 2529) -> (junction 2532)
          ExtraFunctions -> ExtraFunctionsSubMenu [order 2] : SET
          (junction 2532) -> SettingsMenuScreens
          ExtraFunctionsSubMenu -> (junction 2532) : EXIT
        state SetService
          state ServiceMenu
            (history)
            state NextService [commented out]
              en:
              currentState = eStateName.SET_SERVICE_NEXTSERVICE;
            state SetServiceDistance
              state SetServiceDistanceKm
                en:
                currentState = eStateName.SET_SERVICE_DISTANCE_KM;
              state SetServiceDistanceMi
                en:
                currentState = eStateName.SET_SERVICE_DISTANCE_MI;
              (default) -> (junction 1180)
              (junction 1180) -> Flow.ButtonTriggeredMenu.Menu.SetService.ServiceMenu.SetServiceDistance.SetServiceDistanceKm [order 1] : [odoUnits == 0]
              (junction 1180) -> (junction 1183) [order 2]
              (junction 1183) -> Flow.ButtonTriggeredMenu.Menu.SetService.ServiceMenu.SetServiceDistance.SetServiceDistanceMi
            state SetServiceMonths
              en:
              currentState = eStateName.SET_SERVICE_MONTHS_MM;
            (default) -> SetServiceDistance
            SetServiceDistance -> SetServiceMonths [order 2] : UP || DOWN
            SetServiceMonths -> SetServiceDistance [order 2] : UP || DOWN
          state SetServiceDistanceMenu
            state DistanceModifyMenu
              (history)
              state SetServiceDistanceKm
                en:
                currentState = eStateName.CURSOR_ON_KM;
              state SetServiceDistanceMi
                en:
                currentState = eStateName.CURSOR_ON_MI;
            (default) -> (junction 1195)
            Flow.ButtonTriggeredMenu.Menu.SetService.SetServiceDistanceMenu.DistanceModifyMenu.SetServiceDistanceKm -> (junction 1215) [order 2] : DOWN
            (junction 1215) -> (junction 1217) : {BLU_FnDecSrvcDistKM();}
            (junction 1195) -> Flow.ButtonTriggeredMenu.Menu.SetService.SetServiceDistanceMenu.DistanceModifyMenu.SetServiceDistanceKm [order 1] : [odoUnits == 0]
            Flow.ButtonTriggeredMenu.Menu.SetService.SetServiceDistanceMenu.DistanceModifyMenu.SetServiceDistanceKm -> (junction 1205) [order 1] : UP
            (junction 1195) -> (junction 1196) [order 2]
            (junction 1205) -> (junction 1207) : {BLU_FnIncSrvcDistKM();}
            (junction 1207) -> DistanceModifyMenu
            (junction 1217) -> (junction 1207)
            (junction 1211) -> (junction 1207) : {BLU_FnIncSrvcDistMI();}
            (junction 1220) -> (junction 1217) : {BLU_FnDecSrvcDistMI();}
            Flow.ButtonTriggeredMenu.Menu.SetService.SetServiceDistanceMenu.DistanceModifyMenu.SetServiceDistanceMi -> (junction 1211) [order 1] : UP
            (junction 1196) -> Flow.ButtonTriggeredMenu.Menu.SetService.SetServiceDistanceMenu.DistanceModifyMenu.SetServiceDistanceMi
            Flow.ButtonTriggeredMenu.Menu.SetService.SetServiceDistanceMenu.DistanceModifyMenu.SetServiceDistanceMi -> (junction 1220) [order 2] : DOWN
          state SetServiceMonthsMenu
            en:
            currentState = eStateName.CURSON_ON_DATE;
          (default) -> ServiceMenu
          ServiceMenu -> (junction 3549) [order 2] : EXIT
          (junction 3549) -> 3546
          ServiceMenu -> 3546 [order 1] : [duration(set,msec) >=3000]
              | {BLU_FnSaveSrvcChanges();}
          SetServiceDistance -> SetServiceDistanceMenu [order 1] : SET
          SetServiceDistanceMenu -> (junction 3023) : EXIT || SET
          (junction 3023) -> ServiceMenu
          SetServiceMonthsMenu -> (junction 3023) [order 3] : EXIT || SET
          SetServiceMonthsMenu -> (junction 1229) [order 1] : UP
          SetServiceMonths -> SetServiceMonthsMenu [order 1] : SET
          (junction 1229) -> (junction 1231) : {BLU_FnIncSrvcMonths();}
          (junction 1231) -> SetServiceMonthsMenu
          (junction 1237) -> (junction 1231)
          SetServiceMonthsMenu -> (junction 1234) [order 2] : DOWN
          (junction 1234) -> (junction 1237) : {BLU_FnDecSrvcMonths();}
        (junction 2598) -> 2564
        MainSubMenu -> 2564 : EXIT
        NoQS -> (junction 2598) : [after(2,sec)]
        (junction 2147) -> (junction 2234) [order 1] : [quickSelectorUp ==eStateName.QS_UP_RIDE_MODE]
        (junction 2147) -> NoQS [order 2]
        (junction 2425) -> NoQS
        (junction 2234) -> (junction 2233)
        (junction 2151) -> (junction 2147) [order 2]
        (junction 2336) -> (junction 2425) [order 2]
        2561 -> (junction 3141)
        3150 -> 3136
        3134 -> (junction 2471)
        (junction 2471) -> (junction 2472)
        (junction 2151) -> (junction 2238) [order 1] : [quickSelectorUp ==eStateName.QS_UP_ABS_MODE ]
        (junction 2238) -> (junction 2239)
        (junction 2168) -> (junction 2151) [order 2]
        (junction 2168) -> (junction 2243) [order 1] : [quickSelectorUp ==eStateName.QS_UP_MTC ]
        (junction 2243) -> (junction 2244)
        (junction 4035) -> (junction 2168) [order 2]
        Motorcycle -> 3128 [order 3] : SET
        (junction 2233) -> 2650
        (junction 2336) -> (junction 2233) [order 1] : [quickSelectorDown ==eStateName.QS_DOWN_RIDE_MODE]
        (junction 2344) -> (junction 2336) [order 2]
        (junction 2239) -> 2288
        (junction 2344) -> (junction 2239) [order 1] : [quickSelectorDown ==eStateName.QS_DOWN_ABS_MODE ]
        3131 -> (junction 2472)
        (junction 2347) -> (junction 2344) [order 2]
        (junction 2472) -> (junction 2474)
        (junction 2244) -> 2291
        (junction 2347) -> (junction 2244) [order 1] : [quickSelectorDown ==eStateName.QS_DOWN_MTC ]
        (junction 4038) -> (junction 2347) [order 2]
        (junction 4035) -> (junction 4042) [order 1] : [quickSelectorUp ==eStateName.QS_UP_BIKEINFO ]
        (junction 4042) -> (junction 4037)
        (junction 2182) -> (junction 4035) [order 2]
        (junction 4038) -> (junction 4037) [order 1] : [quickSelectorDown ==eStateName.QS_DOWN_BIKEINFO ]
        (junction 4037) -> 4048
        (junction 2350) -> (junction 4038) [order 2]
        BikeInfo -> 3100 [order 3] : SET
        3103 -> (junction 2474)
        (junction 2182) -> (junction 2248) [order 1] : [quickSelectorUp ==eStateName.QS_UP_TRIP1 ]
        (junction 2474) -> (junction 2476)
        (junction 2248) -> (junction 2249)
        (junction 2216) -> (junction 2182) [order 2]
        (junction 2216) -> (junction 2253) [order 1] : [quickSelectorUp ==eStateName.QS_UP_TRIP2 ]
        (junction 2253) -> (junction 2254)
        (junction 2281) -> (junction 2216) [order 2]
        TripInfo -> 3083 [order 3] : SET
        (junction 2350) -> (junction 2249) [order 1] : [quickSelectorDown ==eStateName.QS_DOWN_TRIP1 ]
        (junction 2249) -> 2270
        (junction 2353) -> (junction 2350) [order 2]
        (junction 2353) -> (junction 2254) [order 1] : [quickSelectorDown ==eStateName.QS_DOWN_TRIP2 ]
        3081 -> (junction 2476)
        (junction 2254) -> 2274
        (junction 2356) -> (junction 2353) [order 2]
        (junction 2476) -> (junction 2478)
        (junction 2281) -> (junction 2277) [order 1] : [quickSelectorUp ==eStateName.QS_UP_CRUISECONTROL ]
        (junction 2277) -> (junction 2278)
        (junction 2308) -> (junction 2281) [order 2]
        (junction 2278) -> 2267
        (junction 2356) -> (junction 2278) [order 1] : [quickSelectorDown ==eStateName.QS_DOWN_CRUISECONTROL ]
        CruiseControlMain -> 3073 [order 3] : SET
        (junction 2359) -> (junction 2356) [order 2]
        3071 -> (junction 2478)
        (junction 2478) -> (junction 2481)
        (junction 2308) -> (junction 2306) [order 1] : [quickSelectorUp ==eStateName.QS_UP_NAVIGATION ]
        (junction 2306) -> (junction 2304)
        (junction 2328) -> (junction 2308) [order 2]
        (junction 2359) -> (junction 2304) [order 1] : [quickSelectorDown ==eStateName.QS_DOWN_NAVIGATION ]
        (junction 2304) -> 2666
        3068 -> 3065
        (junction 2362) -> (junction 2359) [order 2]
        3063 -> (junction 2481)
        (junction 2481) -> (junction 2484)
        (junction 2328) -> (junction 2326) [order 1] : [quickSelectorUp ==eStateName.QS_UP_HEATEDGRIPS ]
        (junction 2326) -> (junction 2324)
        (junction 2226) -> (junction 2328) [order 2]
        (junction 2362) -> (junction 2324) [order 1] : [quickSelectorDown ==eStateName.QS_DOWN_HEATEDGRIPS ]
        HeatedGripsMain -> 3053 [order 3] : SET
        (junction 2324) -> 2320
        (junction 2365) -> (junction 2362) [order 2]
        3056 -> (junction 2484)
        (junction 2484) -> (junction 2487)
        (junction 2226) -> (junction 2262) [order 1] : [quickSelectorUp ==eStateName.QS_UP_AUDIO ]
        (junction 2262) -> (junction 2263)
        2569 -> (junction 2226)
        (junction 2263) -> 2222
        (junction 2365) -> (junction 2263) [order 1] : [quickSelectorDown ==eStateName.QS_DOWN_AUDIO ]
        3022 -> 3018
        2566 -> (junction 2365)
        3015 -> (junction 2487)
        (junction 2487) -> (junction 2490)
        3010 -> 2699
        4266 -> 4264
        (junction 2490) -> MainSubMenu
        2715 -> (junction 2490)
        3547 -> SettingsMain
        3012 -> SetService
      state MainScreen
        state RemoteControMode
          en:
          currentState = eStateName.REMOTE_CONTROL_MODE;
          DASH_RCM_Ready_Switch = eButton.pressed;
        state WaitForButton
          en:
          currentState = eStateName.MAIN_SCREEN;
          QuickSelectorDbg = 0;
        WaitForButton -> RemoteControMode [order 4] : [CCU_RCM_Feature == 1 && ...
            | CCU_RCM_Ready_Status == 1]
        RemoteControMode -> WaitForButton : longEXIT
        (default) -> WaitForButton
        2590 -> WaitForButton
        WaitForButton -> (junction 105) [order 1] : SET
        (junction 105) -> 2593 [order 2]
        (junction 105) -> (junction 107) [order 1] : [ECU_SL_LED == 1 && ...
            | ECU_CC_Feature == 0]
            | {DASH_CC_Master_Switch = eButton.pressed;}
        (junction 107) -> WaitForButton
        WaitForButton -> (junction 60) [order 2] : UP
        (junction 70) -> WaitForButton
        WaitForButton -> (junction 84) [order 3] : DOWN
        (junction 60) -> (junction 70) [order 1] : [ECU_SL_Status == 1  && ...
            | ECU_CC_Feature == 0]
            | {DASH_Cc_Resume_Switch  = eButton.pressed;}
        (junction 84) -> (junction 70) [order 1] : [ECU_SL_Status == 1 && ...
            |  ECU_CC_Feature == 0]
            | {DASH_Cc_Set_Switch  = eButton.pressed;}
        (junction 60) -> 2602 [order 2] : [rideMode != eRideMode.track]
        (junction 90) -> (junction 70)
        (junction 84) -> (junction 88) [order 2]
        (junction 88) -> (junction 90) [order 1] : [rideMode == eRideMode.track]
            | {startLapOrLapTimer();}
        (junction 88) -> 2605 [order 2] : [rideMode != eRideMode.track]
      (default) -> MainScreen
      2594 -> 2562
      2603 -> 2570
      2606 -> 2567
      2565 -> 2591
      MainScreen -> 4267 : [hasChangedTo(IgnBattFlg,true)]
      Menu -> MainScreen : [hasChangedTo(INcall,true)]
    state WarningMenu
      state WarningInstruction
        en:
        popUpState = eStateName.POPUP_WARNING_INSTRUCTION;
      (default) -> WarningInstruction
      WarningInstruction -> 3259 : UP || DOWN || SET || EXIT
    state HidePopUp
      en:
      popUpState = eStateName.POPUP_HIDE;
    state CallOperator
      state ActiveCall
        en:
        currentState = eStateName.ACTIVE_CALL;
      state CallInstructionMenu
        en:
        popUpState = eStateName.POPUP_INCALL_INSTRUCTION;
      state AfterPhoneCall
        en:
        currentState = eStateName.AFTER_CALL;
      (default) -> CallInstructionMenu
      ActiveCall -> (junction 3242) [order 2] : UP
          | {BLU_FnCallVolInc();}
      (junction 3242) -> (junction 3249)
      CallInstructionMenu -> ActiveCall [order 1] : [InCallStatus == 2]
      ActiveCall -> (junction 3249) [order 3] : DOWN
          | {BLU_FnCallVolDec();}
      (junction 3249) -> (junction 4209)
      CallInstructionMenu -> (junction 4215) [order 2] : [InCallStatus == 3]
      ActiveCall -> (junction 4215) [order 4] : [InCallStatus == 3]
      (junction 4215) -> AfterPhoneCall
      ActiveCall -> (junction 4209) [order 1] : EXIT
          | {BLU_FnActvCallEXIT();}
      (junction 4209) -> (junction 4212)
      CallInstructionMenu -> (junction 4201) [order 4] : EXIT
      (junction 4203) -> CallInstructionMenu
      CallInstructionMenu -> (junction 4202) [order 3] : SET
      ActiveCall -> (junction 4212) [order 5] : SET
          | {BLU_FnActvCallSET();}
      (junction 4201) -> (junction 4203) : {BLU_FnIncomingCallReject();}
      (junction 4202) -> (junction 4203) : {BLU_FnIncomingCallAnswer();}
      AfterPhoneCall -> 3255 : after(4,sec)
    (default) -> ButtonTriggeredMenu
    ButtonTriggeredMenu -> WarningMenu [order 1] : warning
    3260 -> HidePopUp
    (junction 3265) -> ButtonTriggeredMenu
    HidePopUp -> (junction 3265) : after(2,sec)
    3256 -> (junction 3265)
    ButtonTriggeredMenu -> CallOperator [order 2] : incomingCall
  state PopUpChecker [parallel]
    settings: executionOrder=1
    state CheckWarning [parallel]
      settings: executionOrder=1
      state WarningDefault
      state WarningPopUp
        en:
        send(warning,Flow);
      (default) -> WarningDefault
      WarningDefault -> WarningPopUp : [hasChangedTo(INwarning,true)]
      WarningPopUp -> WarningDefault : after(100,msec)
    state CheckCall [parallel]
      settings: executionOrder=2
      state CallDefault
      state CallPopUp
        en:
        send(incomingCall,Flow);
      (default) -> CallDefault
      CallDefault -> CallPopUp : [hasChangedTo(INcall,true)]
      CallPopUp -> CallDefault : after(100,msec)
    state CheckEndCall [parallel]
      settings: executionOrder=3
      state EndCallDefault
      state EndCallPopUp
        en:
        send(callEnded,Flow);
      (default) -> EndCallDefault
      EndCallDefault -> EndCallPopUp : [hasChangedTo(INcallEnded,true)]
      EndCallPopUp -> EndCallDefault : after(100,msec)
  state ButtonChecker [parallel]
    settings: executionOrder=2
    state CheckUP [parallel]
      settings: executionOrder=1
      state upHigh
        en:
        DASH_RCM_Up_Switch = eButton.pressed;
        en,du:
        upDur = elapsed(sec);
      state upLow
        en:
        DASH_RCM_Up_Switch = eButton.released;
      (default) -> upLow
      upLow -> upHigh : [hasChangedTo(up,true)]
      (junction 1561) -> upLow
      (junction 1564) -> (junction 1561) : {send(UP, Flow);}
      (junction 1559) -> (junction 1564) [order 1] : [upDur*1000>=BLU_UpDtctMin_Tms && ...
          | upDur*1000 <=BLU_UpDtctMax_Tms ]
      upHigh -> (junction 1559) : [hasChangedTo(up,false)]
      (junction 1576) -> (junction 1561)
      (junction 1559) -> (junction 1568) [order 2]
      (junction 1568) -> (junction 1577) [order 1] : [upDur*1000>=BLU_LngUpDtctMin_Tms && ...
          | upDur*1000 <=BLU_LngUpDtctMax_Tms ]
      (junction 1577) -> (junction 1576) : {send(longUP,Flow);}
      (junction 1568) -> (junction 1573) [order 2]
      (junction 1575) -> (junction 1576)
      (junction 1573) -> (junction 1575)
    state CheckDown [parallel]
      settings: executionOrder=2
      state downHigh
        en:
        DASH_RCM_Down_Switch = eButton.pressed;
        en,du:
        downDur = elapsed(sec);
      state downLow
        en:
        DASH_RCM_Down_Switch = eButton.released;
      (default) -> downLow
      downLow -> downHigh : [hasChangedTo(down,true)]
      (junction 1545) -> downLow
      (junction 1552) -> (junction 1545) : {send(DOWN, Flow);}
      (junction 1539) -> (junction 1552) [order 1] : [downDur*1000>=BLU_DwnDtctMin_Tms && ...
          | downDur*1000 <=BLU_DwnDtctMax_Tms ]
      downHigh -> (junction 1539) : [hasChangedTo(down,false)]
      (junction 1556) -> (junction 1545)
      (junction 1539) -> (junction 1543) [order 2]
      (junction 1543) -> (junction 1542) [order 1] : [downDur*1000>=BLU_LngDwnDtctMin_Tms && ...
          | downDur*1000 <=BLU_LngDwnDtctMax_Tms ]
      (junction 1542) -> (junction 1556) : {send(longDOWN,Flow);}
      (junction 1543) -> (junction 1546) [order 2]
      (junction 1555) -> (junction 1556)
      (junction 1546) -> (junction 1555)
    state CheckSet [parallel]
      settings: executionOrder=3
      state setHigh
        en:
        DASH_RCM_Set_Switch = eButton.pressed;
        en,du:
        setDur = elapsed(sec);
      state setLow
        en:
        DASH_RCM_Set_Switch = eButton.released;
      (default) -> ButtonChecker.CheckSet.setLow
      ButtonChecker.CheckSet.setLow -> ButtonChecker.CheckSet.setHigh : [hasChangedTo(set,true)]
      (junction 1507) -> ButtonChecker.CheckSet.setLow
      (junction 1500) -> (junction 1507) : {send(SET,Flow);}
      (junction 1493) -> (junction 1500) [order 1] : [setDur*1000>=BLU_SetDtctMin_Tms && ...
          | setDur*1000 <=BLU_SetDtctMax_Tms ]
      ButtonChecker.CheckSet.setHigh -> (junction 1493) [order 1] : [hasChangedTo(set,false)]
      (junction 1508) -> (junction 1507)
      (junction 1493) -> (junction 1503) [order 2]
      ButtonChecker.CheckSet.setHigh -> (junction 3694) [order 2] : after(3,sec)
      (junction 3694) -> (junction 1505)
      (junction 1503) -> (junction 1505) [order 1] : [setDur*1000>=BLU_LngSetDtctMin_Tms && ...
          | setDur*1000 <=BLU_LngSetDtctMax_Tms ]
      (junction 1505) -> (junction 1508) : {send(longSET,Flow);}
      (junction 1503) -> (junction 1510) [order 2]
      (junction 1512) -> (junction 1508)
      (junction 1510) -> (junction 1512)
    state CheckExit [parallel]
      settings: executionOrder=4
      state exitHigh
        en:
        DASH_RCM_Exit_Switch = eButton.pressed;
        en,du:
        exitDur = elapsed(sec);
      state exitLow
        en:
        DASH_RCM_Exit_Switch = eButton.released;
      (default) -> exitLow
      exitLow -> exitHigh : [hasChangedTo(exitButton,true)]
